simulink library "xbsIndex_r4"  (Simulink 7.1)
(part 8 of 9)

      |     e = regexprep(lasterr, '\n', '\nError: ');
      |     disp(['Error: While running MaskInit code on block ' tmp_gcb ': ' e]);
      |     error(e);
      |   end
      | end
      settings: AttributesFormatString=<< %<shared_memory_name> >>  CopyFcn=xlBlockMoveCallback(gcbh);  DeleteFcn=xlDestroyGui(gcbh);  ModelCloseFcn=xlDestroyGui(gcbh);  PreSaveFcn=xlBlockPreSaveCallback(gcbh);  PostSaveFcn=xlBlockPostSaveCallback(gcbh);  DestroyFcn=xlDestroyGui(gcbh);  OpenFcn=xlOpenGui(gcbh, 'tofifo_gui.xml', @tofifoenablement, @xlDatatypeAction)  CloseFcn=xlDestroyGui(gcbh);  MoveFcn=xlBlockMoveCallback(gcbh);
      mask Help: eval('');xlDoc('-book','sysgen','-topic','To_FIFO');
      mask StyleString: edit,edit,edit,popup(Locally owned|Owned elsewhere),edit,popup(Standard_FIFO|First_Word_Fall_Through),edit,popup(16|32|64|128|256|512|1K|2K|4K|8K|16K|32K|64K|128K|256K),edit,popup(1|2|3|4|5|6|7|8|9|10|11|12|13|14|15|16|17|18),edit,checkbox,edit,checkbox,edit,checkbox,popup(Fixed-point|Floating-point),edit,popup(Signed  (2's comp)|Unsigned|Floating-point),edit,edit,edit,popup(Single),edit,checkbox,edit,popup(Block RAM|Distributed RAM),edit,checkbox,edit,edit,edit,edit,edit,edit,edit,edit,edit
      mask Display:
      | fprintf('','COMMENT: begin icon graphics');
      | patch([0 80 80 0 0 ],[0 0 91 91 0 ],[0.77 0.82 0.91 ]);
      | plot([0 80 80 0 0 ],[0 0 91 91 0 ]);
      | patch([15.525 31.42 42.42 53.42 64.42 42.42 26.525 15.525 ],[57.21 57.21 68.21 57.21 68.21 68.21 68.21 57.21 ],[1 1 1 ]);
      | patch([26.525 42.42 31.42 15.525 26.525 ],[46.21 46.21 57.21 57.21 46.21 ],[0.931 0.946 0.973 ]);
      | patch([15.525 31.42 42.42 26.525 15.525 ],[35.21 35.21 46.21 46.21 35.21 ],[1 1 1 ]);
      | patch([26.525 64.42 53.42 42.42 31.42 15.525 26.525 ],[24.21 24.21 35.21 24.21 35.21 35.21 24.21 ],[0.931 0.946 0.973 ]);
      | fprintf('','COMMENT: end icon graphics');
      | fprintf('','COMMENT: begin icon text');
      | color('black');port_label('input',1,'data_in');
      | color('black');port_label('input',2,'we');
      | color('black');port_label('output',1,'%full');
      | color('black');port_label('output',2,'full');
      | fprintf('','COMMENT: end icon text');
  To Register : S-Function  LoadFcn=xlBlockLoadCallback(gcbh);  FunctionName=sysgen  Parameters=ptable_  EnableBusSupport=off  mask(Xilinx Shared Memory Based To Register Block){infoedit=Register block that writes data to a shared memory register.  Delay of one sample period., shared_memory_name='Bar', init=0, ownership_sgadvanced=, ownership=Locally owned and initialized, explicit_data_type_sgadvanced=, explicit_data_type=off, gui_display_data_type=Fixed-point, arith_type_sgadvanced=, arith_type=Signed  (2's comp), n_bits=16, bin_pt=14, preci_type_sgadvanced=, preci_type=Single, dbl_ovrd_sgadvanced=, dbl_ovrd=off, xl_use_area_sgadvanced=, xl_use_area=off, xl_area=[0,0,0,0,0,0,0], has_advanced_control=0, sggui_pos=-1,-1,-1,-1, block_type=toreg, block_version=, sg_icon_stat=60,56,2,1,white,blue,0,10ab453e,right,,[ ],[ ], sg_mask_display=|, sg_list_contents=, sg_blockgui_xml=}
      mask sg_mask_display=|
      | fprintf('','COMMENT: begin icon graphics');
      | patch([0 60 60 0 0 ],[0 0 56 56 0 ],[0.77 0.82 0.91 ]);
      | plot([0 60 60 0 0 ],[0 0 56 56 0 ]);
      | patch([12.2 23.76 31.76 39.76 47.76 31.76 20.2 12.2 ],[36.88 36.88 44.88 36.88 44.88 44.88 44.88 36.88 ],[1 1 1 ]);
      | patch([20.2 31.76 23.76 12.2 20.2 ],[28.88 28.88 36.88 36.88 28.88 ],[0.931 0.946 0.973 ]);
      | patch([12.2 23.76 31.76 20.2 12.2 ],[20.88 20.88 28.88 28.88 20.88 ],[1 1 1 ]);
      | patch([20.2 47.76 39.76 31.76 23.76 12.2 20.2 ],[12.88 12.88 20.88 12.88 20.88 20.88 12.88 ],[0.931 0.946 0.973 ]);
      | fprintf('','COMMENT: end icon graphics');
      | fprintf('','COMMENT: begin icon text');
      | color('black');port_label('input',1,'din');
      | color('black');port_label('input',2,'en');
      | color('black');port_label('output',1,'dout');
      | fprintf('','COMMENT: end icon text');
      mask prompts: infoedit ""; shared_memory_name "Shared memory name"; init "Initial value"; ownership_sgadvanced ""; ownership "Ownership and initialization"; explicit_data_type_sgadvanced ""; explicit_data_type "Specify explicit output type"; gui_display_data_type ""; arith_type_sgadvanced ""; arith_type "Arithmetic type"; n_bits "Number of bits"; bin_pt "Binary point"; preci_type_sgadvanced ""; preci_type ""; dbl_ovrd_sgadvanced ""; dbl_ovrd "Override with doubles"; xl_use_area_sgadvanced ""; xl_use_area "Define FPGA area for resource estimation"; xl_area "FPGA area [slices, FFs, BRAMs, LUTs, IOBs, emb. mults, TBUFs]"; has_advanced_control ""; sggui_pos ""; block_type ""; block_version ""; sg_icon_stat ""; sg_mask_display ""; sg_list_contents ""; sg_blockgui_xml ""
      mask help: Register block that writes data to a shared memory register. Delay of one sample period.
      mask init:
      | try
      |   tmp_gcb = gcb;
      |   tmp_gcbh = gcbh;
      |   if (strcmp('SysGenIndex',get_param(bdroot(tmp_gcbh),'tag')) && ~isempty(regexp(bdroot(tmp_gcb), '^xbs', 'once')))
      |     return;
      |   end;
      |   xlMungeMaskParams;
      |   block_config = 'sysgen_blockset:toreg_config';
      | 
      |   block_type='toreg';
      | 
      |   serialized_declarations = '{''arith_type''=>''Int'',''bin_pt''=>''Int'',''dbl_ovrd''=>''Int'',''explicit_data_type''=>''Int'',''gui_display_data_type''=>''Int'',''init''=>''Double'',''n_bits''=>''Int'',''ownership''=>''Int'',''preci_type''=>''Int'',''shared_memory_name''=>''String'',''block_type''=>''String''}';
      |   ptable_ = xlblockprep(get_param(tmp_gcb, 'MaskWSVariables'));
      |   try
      |     xlBlockMoveCallback(tmp_gcbh);
      |   catch 
      |      clear global xl_updateicon_recursion_guard;
      |   end;
      | catch
      |   global dbgsysgen;
      |   if(~isempty(dbgsysgen) && dbgsysgen)
      |     e = regexprep(lasterr, '\n', '\nError: ');
      |     disp(['Error: While running MaskInit code on block ' tmp_gcb ': ' e]);
      |     error(e);
      |   end
      | end
      settings: AttributesFormatString=<< %<shared_memory_name> >>  CopyFcn=xlBlockMoveCallback(gcbh);  DeleteFcn=xlDestroyGui(gcbh);  ModelCloseFcn=xlDestroyGui(gcbh);  PreSaveFcn=xlBlockPreSaveCallback(gcbh);  PostSaveFcn=xlBlockPostSaveCallback(gcbh);  DestroyFcn=xlDestroyGui(gcbh);  OpenFcn=xlOpenGui(gcbh, 'toreg_gui.xml', @toregenablement, @xlDatatypeAction)  CloseFcn=xlDestroyGui(gcbh);  MoveFcn=xlBlockMoveCallback(gcbh);
      mask Help: eval('');xlDoc('-book','sysgen','-topic','To_Register');
      mask StyleString: edit,edit,edit,edit,popup(Locally owned and initialized|Owned and initialized elsewhere),edit,checkbox,popup(Fixed-point|Floating-point),edit,popup(Signed  (2's comp)|Unsigned|Floating-point),edit,edit,edit,popup(Single),edit,checkbox,edit,checkbox,edit,edit,edit,edit,edit,edit,edit,edit,edit
      mask Display:
      | fprintf('','COMMENT: begin icon graphics');
      | patch([0 60 60 0 0 ],[0 0 56 56 0 ],[0.77 0.82 0.91 ]);
      | plot([0 60 60 0 0 ],[0 0 56 56 0 ]);
      | patch([12.2 23.76 31.76 39.76 47.76 31.76 20.2 12.2 ],[36.88 36.88 44.88 36.88 44.88 44.88 44.88 36.88 ],[1 1 1 ]);
      | patch([20.2 31.76 23.76 12.2 20.2 ],[28.88 28.88 36.88 36.88 28.88 ],[0.931 0.946 0.973 ]);
      | patch([12.2 23.76 31.76 20.2 12.2 ],[20.88 20.88 28.88 28.88 20.88 ],[1 1 1 ]);
      | patch([20.2 47.76 39.76 31.76 23.76 12.2 20.2 ],[12.88 12.88 20.88 12.88 20.88 20.88 12.88 ],[0.931 0.946 0.973 ]);
      | fprintf('','COMMENT: end icon graphics');
      | fprintf('','COMMENT: begin icon text');
      | color('black');port_label('input',1,'din');
      | color('black');port_label('input',2,'en');
      | color('black');port_label('output',1,'dout');
      | fprintf('','COMMENT: end icon text');
  Toolbar : S-Function  FunctionName=xlpermissive  Parameters=''  EnableBusSupport=off  mask(Xilinx Toolbar Block){infoedit=Toolbar, func=xltoolbar, ShowPortLabels=, has_advanced_control=0, sggui_pos=-1,-1,-1,-1, block_type=toolbar, block_version=, sg_icon_stat=50,54,-1,-1,blue,white,0,07734,right,,[ ],[ ], sg_mask_display=|, sg_list_contents=, sg_blockgui_xml=}
      mask sg_mask_display=|
      | fprintf('','COMMENT: begin icon graphics');
      | patch([0 50 50 0 0 ],[0 0 54 54 0 ],[1 1 1 ]);
      | plot([0 50 50 0 0 ],[0 0 54 54 0 ]);
      | patch([9.425 19.54 26.54 33.54 40.54 26.54 16.425 9.425 ],[34.77 34.77 41.77 34.77 41.77 41.77 41.77 34.77 ],[0.839 0.874 0.937 ]);
      | patch([16.425 26.54 19.54 9.425 16.425 ],[27.77 27.77 34.77 34.77 27.77 ],[0.77 0.82 0.91 ]);
      | patch([9.425 19.54 26.54 16.425 9.425 ],[20.77 20.77 27.77 27.77 20.77 ],[0.839 0.874 0.937 ]);
      | patch([16.425 40.54 33.54 26.54 19.54 9.425 16.425 ],[13.77 13.77 20.77 13.77 20.77 20.77 13.77 ],[0.77 0.82 0.91 ]);
      | fprintf('','COMMENT: end icon graphics');
      | fprintf('','COMMENT: begin icon text');
      | fprintf('','COMMENT: end icon text');
      mask prompts: infoedit ""; func "Launch function"; ShowPortLabels ""; has_advanced_control ""; sggui_pos ""; block_type ""; block_version ""; sg_icon_stat ""; sg_mask_display ""; sg_list_contents ""; sg_blockgui_xml ""
      mask help: Toolbar
      mask init:
      | try
      |   tmp_gcb = gcb;
      |   tmp_gcbh = gcbh;
      |   if (strcmp('SysGenIndex',get_param(bdroot(tmp_gcbh),'tag')) && ~isempty(regexp(bdroot(tmp_gcb), '^xbs', 'once')))
      |     return;
      |   end;
      |   xlMungeMaskParams;
      | 
      |   block_type='toolbar';
      | 
      |   serialized_declarations = '{''block_type''=>''String''}';
      |   ptable_ = xlblockprep(get_param(tmp_gcb, 'MaskWSVariables'));
      |   try
      |     xlBlockMoveCallback(tmp_gcbh);
      |   catch 
      |      clear global xl_updateicon_recursion_guard;
      |   end;
      | catch
      |   global dbgsysgen;
      |   if(~isempty(dbgsysgen) && dbgsysgen)
      |     e = regexprep(lasterr, '\n', '\nError: ');
      |     disp(['Error: While running MaskInit code on block ' tmp_gcb ': ' e]);
      |     error(e);
      |   end
      | end
      settings: CopyFcn=xlBlockMoveCallback(gcbh);  OpenFcn=xltoolbar;  MoveFcn=xlBlockMoveCallback(gcbh);
      mask Help: eval('');xlDoc('-book','sysgen','-topic','Toolbar');
      mask Display:
      | fprintf('','COMMENT: begin icon graphics');
      | patch([0 50 50 0 0 ],[0 0 54 54 0 ],[1 1 1 ]);
      | plot([0 50 50 0 0 ],[0 0 54 54 0 ]);
      | patch([9.425 19.54 26.54 33.54 40.54 26.54 16.425 9.425 ],[34.77 34.77 41.77 34.77 41.77 41.77 41.77 34.77 ],[0.839 0.874 0.937 ]);
      | patch([16.425 26.54 19.54 9.425 16.425 ],[27.77 27.77 34.77 34.77 27.77 ],[0.77 0.82 0.91 ]);
      | patch([9.425 19.54 26.54 16.425 9.425 ],[20.77 20.77 27.77 27.77 20.77 ],[0.839 0.874 0.937 ]);
      | patch([16.425 40.54 33.54 26.54 19.54 9.425 16.425 ],[13.77 13.77 20.77 13.77 20.77 20.77 13.77 ],[0.77 0.82 0.91 ]);
      | fprintf('','COMMENT: end icon graphics');
      | fprintf('','COMMENT: begin icon text');
      | fprintf('','COMMENT: end icon text');
  Up Sample : S-Function  LoadFcn=xlBlockLoadCallback(gcbh);  FunctionName=sysgen  Parameters=ptable_  EnableBusSupport=off  mask(Xilinx Up Sampler Block){infoedit=Up samples input data.  Inserted values  can be zeros or copies of the most recent input sample.<br><br>Hardware notes: No hardware is needed if inserted values are copies of the input sample; otherwise, a mux and single bit flip-flop are used., sample_ratio=2, copy_samples_sgadvanced=, copy_samples=off, en_sgadvanced=, en=off, latency=0, dbl_ovrd_sgadvanced=, dbl_ovrd=off, xl_use_area_sgadvanced=, xl_use_area=off, xl_area=[0,0,0,0,0,0,0], has_advanced_control=0, sggui_pos=-1,-1,-1,-1, block_type=usamp, block_version=, sg_icon_stat=60,54,1,1,white,blue,0,cf641474,right,,[ ],[ ], sg_mask_display=|, sg_list_contents=, sg_blockgui_xml=}
      mask sg_mask_display=|
      | fprintf('','COMMENT: begin icon graphics');
      | patch([0 60 60 0 0 ],[0 0 54 54 0 ],[0.77 0.82 0.91 ]);
      | plot([0 60 60 0 0 ],[0 0 54 54 0 ]);
      | patch([14.425 24.54 31.54 38.54 45.54 31.54 21.425 14.425 ],[34.77 34.77 41.77 34.77 41.77 41.77 41.77 34.77 ],[1 1 1 ]);
      | patch([21.425 31.54 24.54 14.425 21.425 ],[27.77 27.77 34.77 34.77 27.77 ],[0.931 0.946 0.973 ]);
      | patch([14.425 24.54 31.54 21.425 14.425 ],[20.77 20.77 27.77 27.77 20.77 ],[1 1 1 ]);
      | patch([21.425 45.54 38.54 31.54 24.54 14.425 21.425 ],[13.77 13.77 20.77 13.77 20.77 20.77 13.77 ],[0.931 0.946 0.973 ]);
      | fprintf('','COMMENT: end icon graphics');
      | fprintf('','COMMENT: begin icon text');
      |
      |
      | color('black');disp('{\fontsize{14pt}\bf\uparrow}2','texmode','on');
      | fprintf('','COMMENT: end icon text');
      mask prompts: infoedit ""; sample_ratio "Sampling rate (number of output samples per input sample)"; copy_samples_sgadvanced ""; copy_samples "Copy samples (otherwise zeros are inserted)"; en_sgadvanced ""; en "Provide enable port"; dbl_ovrd_sgadvanced ""; dbl_ovrd "Override with doubles"; xl_use_area_sgadvanced ""; xl_use_area "Define FPGA area for resource estimation"; xl_area "FPGA area [slices, FFs, BRAMs, LUTs, IOBs, emb. mults, TBUFs]"; has_advanced_control ""; sggui_pos ""; block_type ""; block_version ""; sg_icon_stat ""; sg_mask_display ""; sg_list_contents ""; sg_blockgui_xml ""
      mask help:
      | Up samples input data.  Inserted values  can be zeros or copies of the most recent input sample.
      |
      | Hardware notes: No hardware is needed if inserted values are copies of the input sample; otherwise, a mux and single bit flip-flop are used.
      mask init:
      | try
      |   tmp_gcb = gcb;
      |   tmp_gcbh = gcbh;
      |   if (strcmp('SysGenIndex',get_param(bdroot(tmp_gcbh),'tag')) && ~isempty(regexp(bdroot(tmp_gcb), '^xbs', 'once')))
      |     return;
      |   end;
      |   xlMungeMaskParams;
      |   block_config = 'sysgen_blockset:Upsample_config';
      | 
      |   block_type='usamp';
      | 
      |   serialized_declarations = '{''copy_samples''=>''Int'',''en''=>''Int'',''latency''=>''Int'',''sample_ratio''=>''Int'',''sim_engine''=>''Int'',''sysgen_root''=>''String'',''block_type''=>''String''}';
      |   xlusamp_init();
      |   ptable_ = xlblockprep(get_param(tmp_gcb, 'MaskWSVariables'));
      |   try
      |     xlBlockMoveCallback(tmp_gcbh);
      |   catch 
      |      clear global xl_updateicon_recursion_guard;
      |   end;
      | catch
      |   global dbgsysgen;
      |   if(~isempty(dbgsysgen) && dbgsysgen)
      |     e = regexprep(lasterr, '\n', '\nError: ');
      |     disp(['Error: While running MaskInit code on block ' tmp_gcb ': ' e]);
      |     error(e);
      |   end
      | end
      settings: CopyFcn=xlBlockMoveCallback(gcbh);  DeleteFcn=xlDestroyGui(gcbh);  ModelCloseFcn=xlDestroyGui(gcbh);  PreSaveFcn=xlBlockPreSaveCallback(gcbh);  PostSaveFcn=xlBlockPostSaveCallback(gcbh);  DestroyFcn=xlDestroyGui(gcbh);  OpenFcn=xlOpenGui(gcbh, 'usamp_gui.xml', @xlmagicenablement, -1)  CloseFcn=xlDestroyGui(gcbh);  MoveFcn=xlBlockMoveCallback(gcbh);
      mask Help: eval('');xlDoc('-book','sysgen','-topic','Up_Sample');
      mask Display:
      | fprintf('','COMMENT: begin icon graphics');
      | patch([0 60 60 0 0 ],[0 0 54 54 0 ],[0.77 0.82 0.91 ]);
      | plot([0 60 60 0 0 ],[0 0 54 54 0 ]);
      | patch([14.425 24.54 31.54 38.54 45.54 31.54 21.425 14.425 ],[34.77 34.77 41.77 34.77 41.77 41.77 41.77 34.77 ],[1 1 1 ]);
      | patch([21.425 31.54 24.54 14.425 21.425 ],[27.77 27.77 34.77 34.77 27.77 ],[0.931 0.946 0.973 ]);
      | patch([14.425 24.54 31.54 21.425 14.425 ],[20.77 20.77 27.77 27.77 20.77 ],[1 1 1 ]);
      | patch([21.425 45.54 38.54 31.54 24.54 14.425 21.425 ],[13.77 13.77 20.77 13.77 20.77 20.77 13.77 ],[0.931 0.946 0.973 ]);
      | fprintf('','COMMENT: end icon graphics');
      | fprintf('','COMMENT: begin icon text');
      | 
      | 
      | color('black');disp('{\fontsize{14pt}\bf\uparrow}2','texmode','on');
      | fprintf('','COMMENT: end icon text');
  "VDMA Interface 4.0 " : S-Function  LoadFcn=xlBlockLoadCallback(gcbh);  FunctionName=sysgen  Parameters=ptable_  EnableBusSupport=off  mask(Xilinx VDMA Interface Block){infoedit=This is a bit-accurate simulation model for multiple AXI VDMA external memory interfaces.  Netlisting will generate the port interface that can be attached to the VDMA IP.  This block is currently in beta., c_mem_size_sgadvanced=, c_mem_size=64MB, c_number_of_vdma_if_sgadvanced=, c_number_of_vdma_if=1, c_stream_if_configuration_1_sgadvanced=, c_stream_if_configuration_1=Master/Slave, c_no_of_frames_1=3, c_use_fsync_1_sgadvanced=, c_use_fsync_1=off, c_flush_on_fsync_1_sgadvanced=, c_flush_on_fsync_1=off, c_use_sg_engine_1_sgadvanced=, c_use_sg_engine_1=off, c_video_prm_read_1_sgadvanced=, c_video_prm_read_1=on, c_m_axis_mm2s_data_width_1_sgadvanced=, c_m_axis_mm2s_data_width_1=32, c_mm2s_linebuffer_depth_1_sgadvanced=, c_mm2s_linebuffer_depth_1=0, c_mm2s_linebuffer_threshold_1=1, c_s_axis_s2mm_data_width_1_sgadvanced=, c_s_axis_s2mm_data_width_1=32, c_s2mm_linebuffer_depth_1_sgadvanced=, c_s2mm_linebuffer_depth_1=0, c_s2mm_linebuffer_threshold_1=1, c_stream_if_configuration_2_sgadvanced=, c_stream_if_configuration_2=Master/Slave, c_no_of_frames_2=3, c_use_fsync_2_sgadvanced=, c_use_fsync_2=off, c_flush_on_fsync_2_sgadvanced=, c_flush_on_fsync_2=off, c_use_sg_engine_2_sgadvanced=, c_use_sg_engine_2=off, c_video_prm_read_2_sgadvanced=, c_video_prm_read_2=on, c_m_axis_mm2s_data_width_2_sgadvanced=, c_m_axis_mm2s_data_width_2=32, c_mm2s_linebuffer_depth_2_sgadvanced=, c_mm2s_linebuffer_depth_2=0, c_mm2s_linebuffer_threshold_2=1, c_s_axis_s2mm_data_width_2_sgadvanced=, c_s_axis_s2mm_data_width_2=32, c_s2mm_linebuffer_depth_2_sgadvanced=, c_s2mm_linebuffer_depth_2=0, c_s2mm_linebuffer_threshold_2=1, c_stream_if_configuration_3_sgadvanced=, c_stream_if_configuration_3=Master/Slave, c_no_of_frames_3=3, c_use_fsync_3_sgadvanced=, c_use_fsync_3=off, c_flush_on_fsync_3_sgadvanced=, c_flush_on_fsync_3=off, c_use_sg_engine_3_sgadvanced=, c_use_sg_engine_3=off, c_video_prm_read_3_sgadvanced=, c_video_prm_read_3=on, c_m_axis_mm2s_data_width_3_sgadvanced=, c_m_axis_mm2s_data_width_3=32, c_mm2s_linebuffer_depth_3_sgadvanced=, c_mm2s_linebuffer_depth_3=0, c_mm2s_linebuffer_threshold_3=1, c_s_axis_s2mm_data_width_3_sgadvanced=, c_s_axis_s2mm_data_width_3=32, c_s2mm_linebuffer_depth_3_sgadvanced=, c_s2mm_linebuffer_depth_3=0, c_s2mm_linebuffer_threshold_3=1, c_stream_if_configuration_4_sgadvanced=, c_stream_if_configuration_4=Master/Slave, c_no_of_frames_4=3, c_use_fsync_4_sgadvanced=, c_use_fsync_4=off, c_flush_on_fsync_4_sgadvanced=, c_flush_on_fsync_4=off, c_use_sg_engine_4_sgadvanced=, c_use_sg_engine_4=off, c_video_prm_read_4_sgadvanced=, c_video_prm_read_4=on, c_m_axis_mm2s_data_width_4_sgadvanced=, c_m_axis_mm2s_data_width_4=32, c_mm2s_linebuffer_depth_4_sgadvanced=, c_mm2s_linebuffer_depth_4=0, c_mm2s_linebuffer_threshold_4=1, c_s_axis_s2mm_data_width_4_sgadvanced=, c_s_axis_s2mm_data_width_4=32, c_s2mm_linebuffer_depth_4_sgadvanced=, c_s2mm_linebuffer_depth_4=0, c_s2mm_linebuffer_threshold_4=1, simulation_model='emi:EMIModel', has_advanced_control=0, sggui_pos=-1,-1,-1,-1, block_type=vdma, block_version=, sg_icon_stat=335,744,14,19,white,yellow,0,358287e6,right,,[2 2 2 2 2 2 2 2 3 3 3 3 4 1 ],[2 2 2 2 2 2 2 2 3 4 4 4 4 1 1 1 1 1 1 ], sg_mask_display=|, sg_list_contents=, sg_blockgui_xml=}
      mask sg_mask_display=|
      | fprintf('','COMMENT: begin icon graphics');
      | patch([0 0 5 5 ],[744 323 323 744 ],[7.375000e-001 7.225000e-001 5.125000e-001 ]);
      | patch([0 0 5 5 ],[306 103 103 306 ],[5.250000e-001 5.150000e-001 3.750000e-001 ]);
      | patch([0 0 5 5 ],[86 48 48 86 ],[3.125000e-001 3.075000e-001 2.375000e-001 ]);
      | patch([0 0 5 5 ],[31 -7 -7 31 ],[9.500000e-001 9.300000e-001 6.500000e-001 ]);
      | patch([330 330 335 335 ],[744 438 438 744 ],[7.375000e-001 7.225000e-001 5.125000e-001 ]);
      | patch([330 330 335 335 ],[426 398 398 426 ],[5.250000e-001 5.150000e-001 3.750000e-001 ]);
      | patch([330 330 335 335 ],[386 238 238 386 ],[3.125000e-001 3.075000e-001 2.375000e-001 ]);
      | patch([330 330 335 335 ],[226 -2 -2 226 ],[9.500000e-001 9.300000e-001 6.500000e-001 ]);
      | patch([5 329 329 5 5 ],[0 0 744 744 0 ],[9.500000e-001 9.300000e-001 6.500000e-001 ]);
      | plot([5 329 329 5 5 ],[0 0 744 744 0 ]);
      |
      |
      | patch([62.425 130.34 177.34 224.34 271.34 177.34 109.425 62.425 ],[424.17 424.17 471.17 424.17 471.17 471.17 471.17 424.17 ],[1 1 1 ]);
      | patch([109.425 177.34 130.34 62.425 109.425 ],[377.17 377.17 424.17 424.17 377.17 ],[0.985 0.979 0.895 ]);
      | patch([62.425 130.34 177.34 109.425 62.425 ],[330.17 330.17 377.17 377.17 330.17 ],[1 1 1 ]);
      | patch([109.425 271.34 224.34 177.34 130.34 62.425 109.425 ],[283.17 283.17 330.17 283.17 330.17 330.17 283.17 ],[0.985 0.979 0.895 ]);
      | fprintf('','COMMENT: end icon graphics');
      | fprintf('','COMMENT: begin icon text');
      | color('black');port_label('input',1,'  vdma_1_s_axi_lite_awvalid  ');
      | color('black');port_label('input',2,'  vdma_1_s_axi_lite_awaddr  ');
      | color('black');port_label('input',3,'  vdma_1_s_axi_lite_wvalid  ');
      | color('black');port_label('input',4,'  vdma_1_s_axi_lite_wdata  ');
      | color('black');port_label('input',5,'  vdma_1_s_axi_lite_bready  ');
      | color('black');port_label('input',6,'  vdma_1_s_axi_lite_arvalid  ');
      | color('black');port_label('input',7,'  vdma_1_s_axi_lite_araddr  ');
      | color('black');port_label('input',8,'  vdma_1_s_axi_lite_rready  ');
      | color('black');port_label('input',9,'  vdma_1_s_axis_s2mm_tdata  ');
      | color('black');port_label('input',10,'  vdma_1_s_axis_s2mm_tkeep  ');
      | color('black');port_label('input',11,'  vdma_1_s_axis_s2mm_tvalid  ');
      | color('black');port_label('input',12,'  vdma_1_s_axis_s2mm_tlast  ');
      | color('black');port_label('input',13,'  vdma_1_m_axis_mm2s_tready  ');
      | color('black');port_label('input',14,'  vdma_1_axi_resetn  ');
      | color('black');port_label('output',1,'  vdma_1_s_axi_lite_awready  ');
      | color('black');port_label('output',2,'  vdma_1_s_axi_lite_wready  ');
      | color('black');port_label('output',3,'  vdma_1_s_axi_lite_bresp  ');
      | color('black');port_label('output',4,'  vdma_1_s_axi_lite_bvalid  ');
      | color('black');port_label('output',5,'  vdma_1_s_axi_lite_arready  ');
      | color('black');port_label('output',6,'  vdma_1_s_axi_lite_rvalid  ');
      | color('black');port_label('output',7,'  vdma_1_s_axi_lite_rdata  ');
      | color('black');port_label('output',8,'  vdma_1_s_axi_lite_rresp  ');
      | color('black');port_label('output',9,'  vdma_1_s_axis_s2mm_tready  ');
      | color('black');port_label('output',10,'  vdma_1_m_axis_mm2s_tdata  ');
      | color('black');port_label('output',11,'  vdma_1_m_axis_mm2s_tkeep  ');
      | color('black');port_label('output',12,'  vdma_1_m_axis_mm2s_tvalid  ');
      | color('black');port_label('output',13,'  vdma_1_m_axis_mm2s_tlast  ');
      | color('black');port_label('output',14,'  vdma_1_mm2s_introut  ');
      | color('black');port_label('output',15,'  vdma_1_mm2s_fsync_out  ');
      | color('black');port_label('output',16,'  vdma_1_mm2s_prmtr_update  ');
      | color('black');port_label('output',17,'  vdma_1_s2mm_introut  ');
      | color('black');port_label('output',18,'  vdma_1_s2mm_fsync_out  ');
      | color('black');port_label('output',19,'  vdma_1_s2mm_prmtr_update  ');
      | fprintf('','COMMENT: end icon text');
      mask prompts: infoedit ""; c_mem_size_sgadvanced ""; c_mem_size "Memory size"; c_number_of_vdma_if_sgadvanced ""; c_number_of_vdma_if "Number of VDMA interfaces"; c_stream_if_configuration_1_sgadvanced ""; c_stream_if_configuration_1 "Stream interface"; c_no_of_frames_1 "Number of frame stores [1..16]"; c_use_fsync_1_sgadvanced ""; c_use_fsync_1 "Use external frame sync"; c_flush_on_fsync_1_sgadvanced ""; c_flush_on_fsync_1 "Flush on frame sync"; c_use_sg_engine_1_sgadvanced ""; c_use_sg_engine_1 "Use Scatter Gather Engine"; c_video_prm_read_1_sgadvanced ""; c_video_prm_read_1 "Use Video Parameter Read for Direct Mode"; c_m_axis_mm2s_data_width_1_sgadvanced ""; c_m_axis_mm2s_data_width_1 "Data width"; c_mm2s_linebuffer_depth_1_sgadvanced ""; c_mm2s_linebuffer_depth_1 "Depth"; c_mm2s_linebuffer_threshold_1 "Almost empty threshold [1..65536]"; c_s_axis_s2mm_data_width_1_sgadvanced ""; c_s_axis_s2mm_data_width_1 "Data width"; c_s2mm_linebuffer_depth_1_sgadvanced ""; c_s2mm_linebuffer_depth_1 "Depth"; c_s2mm_linebuffer_threshold_1 "Almost full threshold [1..65536]"; c_stream_if_configuration_2_sgadvanced ""; c_stream_if_configuration_2 "Stream interface"; c_no_of_frames_2 "Number of frame stores [1..16]"; c_use_fsync_2_sgadvanced ""; c_use_fsync_2 "Use external frame sync"; c_flush_on_fsync_2_sgadvanced ""; c_flush_on_fsync_2 "Flush on frame sync"; c_use_sg_engine_2_sgadvanced ""; c_use_sg_engine_2 "Use Scatter Gather Engine"; c_video_prm_read_2_sgadvanced ""; c_video_prm_read_2 "Use Video Parameter Read for Direct Mode"; c_m_axis_mm2s_data_width_2_sgadvanced ""; c_m_axis_mm2s_data_width_2 "Data width"; c_mm2s_linebuffer_depth_2_sgadvanced ""; c_mm2s_linebuffer_depth_2 "Depth"; c_mm2s_linebuffer_threshold_2 "Almost empty threshold [1..65536]"; c_s_axis_s2mm_data_width_2_sgadvanced ""; c_s_axis_s2mm_data_width_2 "Data width"; c_s2mm_linebuffer_depth_2_sgadvanced ""; c_s2mm_linebuffer_depth_2 "Depth"; c_s2mm_linebuffer_threshold_2 "Almost full threshold [1..65536]"; c_stream_if_configuration_3_sgadvanced ""; c_stream_if_configuration_3 "Stream interface"; c_no_of_frames_3 "Number of frame stores [1..16]"; c_use_fsync_3_sgadvanced ""; c_use_fsync_3 "Use external frame sync"; c_flush_on_fsync_3_sgadvanced ""; c_flush_on_fsync_3 "Flush on frame sync"; c_use_sg_engine_3_sgadvanced ""; c_use_sg_engine_3 "Use Scatter Gather Engine"; c_video_prm_read_3_sgadvanced ""; c_video_prm_read_3 "Use Video Parameter Read for Direct Mode"; c_m_axis_mm2s_data_width_3_sgadvanced ""; c_m_axis_mm2s_data_width_3 "Data width"; c_mm2s_linebuffer_depth_3_sgadvanced ""; c_mm2s_linebuffer_depth_3 "Depth"; c_mm2s_linebuffer_threshold_3 "Almost empty threshold [1..65536]"; c_s_axis_s2mm_data_width_3_sgadvanced ""; c_s_axis_s2mm_data_width_3 "Data width"; c_s2mm_linebuffer_depth_3_sgadvanced ""; c_s2mm_linebuffer_depth_3 "Depth"; c_s2mm_linebuffer_threshold_3 "Almost full threshold [1..65536]"; c_stream_if_configuration_4_sgadvanced ""; c_stream_if_configuration_4 "Stream interface"; c_no_of_frames_4 "Number of frame stores [1..16]"; c_use_fsync_4_sgadvanced ""; c_use_fsync_4 "Use external frame sync"; c_flush_on_fsync_4_sgadvanced ""; c_flush_on_fsync_4 "Flush on frame sync"; c_use_sg_engine_4_sgadvanced ""; c_use_sg_engine_4 "Use Scatter Gather Engine"; c_video_prm_read_4_sgadvanced ""; c_video_prm_read_4 "Use Video Parameter Read for Direct Mode"; c_m_axis_mm2s_data_width_4_sgadvanced ""; c_m_axis_mm2s_data_width_4 "Data width"; c_mm2s_linebuffer_depth_4_sgadvanced ""; c_mm2s_linebuffer_depth_4 "Depth"; c_mm2s_linebuffer_threshold_4 "Almost empty threshold [1..65536]"; c_s_axis_s2mm_data_width_4_sgadvanced ""; c_s_axis_s2mm_data_width_4 "Data width"; c_s2mm_linebuffer_depth_4_sgadvanced ""; c_s2mm_linebuffer_depth_4 "Depth"; c_s2mm_linebuffer_threshold_4 "Almost full threshold [1..65536]"; simulation_model ""; has_advanced_control ""; sggui_pos ""; block_type ""; block_version ""; sg_icon_stat ""; sg_mask_display ""; sg_list_contents ""; sg_blockgui_xml ""
      mask help: This is a bit-accurate simulation model for multiple AXI VDMA external memory interfaces. Netlisting will generate the port interface that can be attached to the VDMA IP. This block is currently in beta.
      mask init:
      | try
      |   tmp_gcb = gcb;
      |   tmp_gcbh = gcbh;
      |   if (strcmp('SysGenIndex',get_param(bdroot(tmp_gcbh),'tag')) && ~isempty(regexp(bdroot(tmp_gcb), '^xbs', 'once')))
      |     return;
      |   end;
      |   xlMungeMaskParams;
      |   block_config = 'emi:emi_all_interfaces_config';
      | 
      |   block_type='vdma';
      | 
      |   serialized_declarations = '{''c_flush_on_fsync_1''=>''Int'',''c_flush_on_fsync_2''=>''Int'',''c_flush_on_fsync_3''=>''Int'',''c_flush_on_fsync_4''=>''Int'',''c_m_axis_mm2s_data_width_1''=>''Int'',''c_m_axis_mm2s_data_width_2''=>''Int'',''c_m_axis_mm2s_data_width_3''=>''Int'',''c_m_axis_mm2s_data_width_4''=>''Int'',''c_mem_size''=>''Int'',''c_mm2s_linebuffer_depth_1''=>''Int'',''c_mm2s_linebuffer_depth_2''=>''Int'',''c_mm2s_linebuffer_depth_3''=>''Int'',''c_mm2s_linebuffer_depth_4''=>''Int'',''c_mm2s_linebuffer_threshold_1''=>''Int'',''c_mm2s_linebuffer_threshold_2''=>''Int'',''c_mm2s_linebuffer_threshold_3''=>''Int'',''c_mm2s_linebuffer_threshold_4''=>''Int'',''c_no_of_frames_1''=>''Int'',''c_no_of_frames_2''=>''Int'',''c_no_of_frames_3''=>''Int'',''c_no_of_frames_4''=>''Int'',''c_number_of_vdma_if''=>''Int'',''c_s2mm_linebuffer_depth_1''=>''Int'',''c_s2mm_linebuffer_depth_2''=>''Int'',''c_s2mm_linebuffer_depth_3''=>''Int'',''c_s2mm_linebuffer_depth_4''=>''Int'',''c_s2mm_linebuffer_threshold_1''=>''Int'',''c_s2mm_linebuffer_threshold_2''=>''Int'',''c_s2mm_linebuffer_threshold_3''=>''Int'',''c_s2mm_linebuffer_threshold_4''=>''Int'',''c_s_axis_s2mm_data_width_1''=>''Int'',''c_s_axis_s2mm_data_width_2''=>''Int'',''c_s_axis_s2mm_data_width_3''=>''Int'',''c_s_axis_s2mm_data_width_4''=>''Int'',''c_stream_if_configuration_1''=>''Int'',''c_stream_if_configuration_2''=>''Int'',''c_stream_if_configuration_3''=>''Int'',''c_stream_if_configuration_4''=>''Int'',''c_use_fsync_1''=>''Int'',''c_use_fsync_2''=>''Int'',''c_use_fsync_3''=>''Int'',''c_use_fsync_4''=>''Int'',''c_use_sg_engine_1''=>''Int'',''c_use_sg_engine_2''=>''Int'',''c_use_sg_engine_3''=>''Int'',''c_use_sg_engine_4''=>''Int'',''c_video_prm_read_1''=>''Int'',''c_video_prm_read_2''=>''Int'',''c_video_prm_read_3''=>''Int'',''c_video_prm_read_4''=>''Int'',''simulation_model''=>''String'',''block_type''=>''String''}';
      |   ptable_ = xlblockprep(get_param(tmp_gcb, 'MaskWSVariables'));
      |   try
      |     xlBlockMoveCallback(tmp_gcbh);
      |   catch 
      |      clear global xl_updateicon_recursion_guard;
      |   end;
      | catch
      |   global dbgsysgen;
      |   if(~isempty(dbgsysgen) && dbgsysgen)
      |     e = regexprep(lasterr, '\n', '\nError: ');
      |     disp(['Error: While running MaskInit code on block ' tmp_gcb ': ' e]);
      |     error(e);
      |   end
      | end
      settings: CopyFcn=xlBlockMoveCallback(gcbh);  DeleteFcn=xlDestroyGui(gcbh);  ModelCloseFcn=xlDestroyGui(gcbh);  PreSaveFcn=xlBlockPreSaveCallback(gcbh);  PostSaveFcn=xlBlockPostSaveCallback(gcbh);  DestroyFcn=xlDestroyGui(gcbh);  OpenFcn=xlOpenGui(gcbh, 'vdma_gui.xml', @xlEMIEnablement, @xlEMIaction)  CloseFcn=xlDestroyGui(gcbh);  MoveFcn=xlBlockMoveCallback(gcbh);
      mask Help: eval('');xlDoc('-book','sysgen','-topic','VDMA_Interface_4_0');
      mask StyleString: edit,edit,popup(16MB|32MB|64MB|128MB|256MB|512MB|1GB|2GB),edit,popup(1|2|3|4),edit,popup(Master/Slave|Master|Slave),edit,edit,checkbox,edit,checkbox,edit,checkbox,edit,checkbox,edit,popup(8|16|32|64|128|256|512|1024),edit,popup(0|1|2|4|8|16|32|64|128|256|512|1024|2048|4096|8192|16384|32768|65536),edit,edit,popup(8|16|32|64|128|256|512|1024),edit,popup(0|1|2|4|8|16|32|64|128|256|512|1024|2048|4096|8192|16384|32768|65536),edit,edit,popup(Master/Slave|Master|Slave),edit,edit,checkbox,edit,checkbox,edit,checkbox,edit,checkbox,edit,popup(8|16|32|64|128|256|512|1024),edit,popup(0|1|2|4|8|16|32|64|128|256|512|1024|2048|4096|8192|16384|32768|65536),edit,edit,popup(8|16|32|64|128|256|512|1024),edit,popup(0|1|2|4|8|16|32|64|128|256|512|1024|2048|4096|8192|16384|32768|65536),edit,edit,popup(Master/Slave|Master|Slave),edit,edit,checkbox,edit,checkbox,edit,checkbox,edit,checkbox,edit,popup(8|16|32|64|128|256|512|1024),edit,popup(0|1|2|4|8|16|32|64|128|256|512|1024|2048|4096|8192|16384|32768|65536),edit,edit,popup(8|16|32|64|128|256|512|1024),edit,popup(0|1|2|4|8|16|32|64|128|256|512|1024|2048|4096|8192|16384|32768|65536),edit,edit,popup(Master/Slave|Master|Slave),edit,edit,checkbox,edit,checkbox,edit,checkbox,edit,checkbox,edit,popup(8|16|32|64|128|256|512|1024),edit,popup(0|1|2|4|8|16|32|64|128|256|512|1024|2048|4096|8192|16384|32768|65536),edit,edit,popup(8|16|32|64|128|256|512|1024),edit,popup(0|1|2|4|8|16|32|64|128|256|512|1024|2048|4096|8192|16384|32768|65536),edit,edit,edit,edit,edit,edit,edit,edit,edit,edit
      mask Display:
      | fprintf('','COMMENT: begin icon graphics');
      | patch([0 0 5 5 ],[744 323 323 744 ],[7.375000e-001 7.225000e-001 5.125000e-001 ]);
      | patch([0 0 5 5 ],[306 103 103 306 ],[5.250000e-001 5.150000e-001 3.750000e-001 ]);
      | patch([0 0 5 5 ],[86 48 48 86 ],[3.125000e-001 3.075000e-001 2.375000e-001 ]);
      | patch([0 0 5 5 ],[31 -7 -7 31 ],[9.500000e-001 9.300000e-001 6.500000e-001 ]);
      | patch([330 330 335 335 ],[744 438 438 744 ],[7.375000e-001 7.225000e-001 5.125000e-001 ]);
      | patch([330 330 335 335 ],[426 398 398 426 ],[5.250000e-001 5.150000e-001 3.750000e-001 ]);
      | patch([330 330 335 335 ],[386 238 238 386 ],[3.125000e-001 3.075000e-001 2.375000e-001 ]);
      | patch([330 330 335 335 ],[226 -2 -2 226 ],[9.500000e-001 9.300000e-001 6.500000e-001 ]);
      | patch([5 329 329 5 5 ],[0 0 744 744 0 ],[9.500000e-001 9.300000e-001 6.500000e-001 ]);
      | plot([5 329 329 5 5 ],[0 0 744 744 0 ]);
      | 
      | 
      | patch([62.425 130.34 177.34 224.34 271.34 177.34 109.425 62.425 ],[424.17 424.17 471.17 424.17 471.17 471.17 471.17 424.17 ],[1 1 1 ]);
      | patch([109.425 177.34 130.34 62.425 109.425 ],[377.17 377.17 424.17 424.17 377.17 ],[0.985 0.979 0.895 ]);
      | patch([62.425 130.34 177.34 109.425 62.425 ],[330.17 330.17 377.17 377.17 330.17 ],[1 1 1 ]);
      | patch([109.425 271.34 224.34 177.34 130.34 62.425 109.425 ],[283.17 283.17 330.17 283.17 330.17 330.17 283.17 ],[0.985 0.979 0.895 ]);
      | fprintf('','COMMENT: end icon graphics');
      | fprintf('','COMMENT: begin icon text');
      | color('black');port_label('input',1,'  vdma_1_s_axi_lite_awvalid  ');
      | color('black');port_label('input',2,'  vdma_1_s_axi_lite_awaddr  ');
      | color('black');port_label('input',3,'  vdma_1_s_axi_lite_wvalid  ');
      | color('black');port_label('input',4,'  vdma_1_s_axi_lite_wdata  ');
      | color('black');port_label('input',5,'  vdma_1_s_axi_lite_bready  ');
      | color('black');port_label('input',6,'  vdma_1_s_axi_lite_arvalid  ');
      | color('black');port_label('input',7,'  vdma_1_s_axi_lite_araddr  ');
      | color('black');port_label('input',8,'  vdma_1_s_axi_lite_rready  ');
      | color('black');port_label('input',9,'  vdma_1_s_axis_s2mm_tdata  ');
      | color('black');port_label('input',10,'  vdma_1_s_axis_s2mm_tkeep  ');
      | color('black');port_label('input',11,'  vdma_1_s_axis_s2mm_tvalid  ');
      | color('black');port_label('input',12,'  vdma_1_s_axis_s2mm_tlast  ');
      | color('black');port_label('input',13,'  vdma_1_m_axis_mm2s_tready  ');
      | color('black');port_label('input',14,'  vdma_1_axi_resetn  ');
      | color('black');port_label('output',1,'  vdma_1_s_axi_lite_awready  ');
      | color('black');port_label('output',2,'  vdma_1_s_axi_lite_wready  ');
      | color('black');port_label('output',3,'  vdma_1_s_axi_lite_bresp  ');
      | color('black');port_label('output',4,'  vdma_1_s_axi_lite_bvalid  ');
      | color('black');port_label('output',5,'  vdma_1_s_axi_lite_arready  ');
      | color('black');port_label('output',6,'  vdma_1_s_axi_lite_rvalid  ');
      | color('black');port_label('output',7,'  vdma_1_s_axi_lite_rdata  ');
      | color('black');port_label('output',8,'  vdma_1_s_axi_lite_rresp  ');
      | color('black');port_label('output',9,'  vdma_1_s_axis_s2mm_tready  ');
      | color('black');port_label('output',10,'  vdma_1_m_axis_mm2s_tdata  ');
      | color('black');port_label('output',11,'  vdma_1_m_axis_mm2s_tkeep  ');
      | color('black');port_label('output',12,'  vdma_1_m_axis_mm2s_tvalid  ');
      | color('black');port_label('output',13,'  vdma_1_m_axis_mm2s_tlast  ');
      | color('black');port_label('output',14,'  vdma_1_mm2s_introut  ');
      | color('black');port_label('output',15,'  vdma_1_mm2s_fsync_out  ');
      | color('black');port_label('output',16,'  vdma_1_mm2s_prmtr_update  ');
      | color('black');port_label('output',17,'  vdma_1_s2mm_introut  ');
      | color('black');port_label('output',18,'  vdma_1_s2mm_fsync_out  ');
      | color('black');port_label('output',19,'  vdma_1_s2mm_prmtr_update  ');
      | fprintf('','COMMENT: end icon text');
  "VDMA Interface 5.0 " : S-Function  LoadFcn=xlBlockLoadCallback(gcbh);  FunctionName=sysgen  Parameters=ptable_  EnableBusSupport=off  mask(Xilinx VDMA Interface 5.0 Block){infoedit=This is a bit-accurate simulation model for multiple AXI VDMA external memory interfaces.  Netlisting will generate the port interface that can be attached to the VDMA IP.  This block is currently in beta., c_mem_size_sgadvanced=, c_mem_size=64MB, c_number_of_vdma_if_sgadvanced=, c_number_of_vdma_if=1, c_stream_if_configuration_1_sgadvanced=, c_stream_if_configuration_1=Master/Slave, c_no_of_frames_1=3, c_use_fsync_1_sgadvanced=, c_use_fsync_1=off, c_flush_on_fsync_1_sgadvanced=, c_flush_on_fsync_1=off, c_use_sg_engine_1_sgadvanced=, c_use_sg_engine_1=off, c_video_prm_read_1_sgadvanced=, c_video_prm_read_1=on, c_m_axis_mm2s_data_width_1_sgadvanced=, c_m_axis_mm2s_data_width_1=32, c_m_axis_mm2s_frame_sync_tuser_1_sgadvanced=, c_m_axis_mm2s_frame_sync_tuser_1=off, c_mm2s_linebuffer_depth_1_sgadvanced=, c_mm2s_linebuffer_depth_1=0, c_mm2s_linebuffer_threshold_1=1, c_s_axis_s2mm_data_width_1_sgadvanced=, c_s_axis_s2mm_data_width_1=32, c_s_axis_s2mm_frame_sync_tuser_1_sgadvanced=, c_s_axis_s2mm_frame_sync_tuser_1=off, c_s2mm_linebuffer_depth_1_sgadvanced=, c_s2mm_linebuffer_depth_1=0, c_s2mm_linebuffer_threshold_1=1, c_stream_if_configuration_2_sgadvanced=, c_stream_if_configuration_2=Master/Slave, c_no_of_frames_2=3, c_use_fsync_2_sgadvanced=, c_use_fsync_2=off, c_flush_on_fsync_2_sgadvanced=, c_flush_on_fsync_2=off, c_use_sg_engine_2_sgadvanced=, c_use_sg_engine_2=off, c_video_prm_read_2_sgadvanced=, c_video_prm_read_2=on, c_m_axis_mm2s_data_width_2_sgadvanced=, c_m_axis_mm2s_data_width_2=32, c_m_axis_mm2s_frame_sync_tuser_2_sgadvanced=, c_m_axis_mm2s_frame_sync_tuser_2=off, c_mm2s_linebuffer_depth_2_sgadvanced=, c_mm2s_linebuffer_depth_2=0, c_mm2s_linebuffer_threshold_2=1, c_s_axis_s2mm_data_width_2_sgadvanced=, c_s_axis_s2mm_data_width_2=32, c_s_axis_s2mm_frame_sync_tuser_2_sgadvanced=, c_s_axis_s2mm_frame_sync_tuser_2=off, c_s2mm_linebuffer_depth_2_sgadvanced=, c_s2mm_linebuffer_depth_2=0, c_s2mm_linebuffer_threshold_2=1, c_stream_if_configuration_3_sgadvanced=, c_stream_if_configuration_3=Master/Slave, c_no_of_frames_3=3, c_use_fsync_3_sgadvanced=, c_use_fsync_3=off, c_flush_on_fsync_3_sgadvanced=, c_flush_on_fsync_3=off, c_use_sg_engine_3_sgadvanced=, c_use_sg_engine_3=off, c_video_prm_read_3_sgadvanced=, c_video_prm_read_3=on, c_m_axis_mm2s_data_width_3_sgadvanced=, c_m_axis_mm2s_data_width_3=32, c_m_axis_mm2s_frame_sync_tuser_3_sgadvanced=, c_m_axis_mm2s_frame_sync_tuser_3=off, c_mm2s_linebuffer_depth_3_sgadvanced=, c_mm2s_linebuffer_depth_3=0, c_mm2s_linebuffer_threshold_3=1, c_s_axis_s2mm_data_width_3_sgadvanced=, c_s_axis_s2mm_data_width_3=32, c_s_axis_s2mm_frame_sync_tuser_3_sgadvanced=, c_s_axis_s2mm_frame_sync_tuser_3=off, c_s2mm_linebuffer_depth_3_sgadvanced=, c_s2mm_linebuffer_depth_3=0, c_s2mm_linebuffer_threshold_3=1, c_stream_if_configuration_4_sgadvanced=, c_stream_if_configuration_4=Master/Slave, c_no_of_frames_4=3, c_use_fsync_4_sgadvanced=, c_use_fsync_4=off, c_flush_on_fsync_4_sgadvanced=, c_flush_on_fsync_4=off, c_use_sg_engine_4_sgadvanced=, c_use_sg_engine_4=off, c_video_prm_read_4_sgadvanced=, c_video_prm_read_4=on, c_m_axis_mm2s_data_width_4_sgadvanced=, c_m_axis_mm2s_data_width_4=32, c_m_axis_mm2s_frame_sync_tuser_4_sgadvanced=, c_m_axis_mm2s_frame_sync_tuser_4=off, c_mm2s_linebuffer_depth_4_sgadvanced=, c_mm2s_linebuffer_depth_4=0, c_mm2s_linebuffer_threshold_4=1, c_s_axis_s2mm_data_width_4_sgadvanced=, c_s_axis_s2mm_data_width_4=32, c_s_axis_s2mm_frame_sync_tuser_4_sgadvanced=, c_s_axis_s2mm_frame_sync_tuser_4=off, c_s2mm_linebuffer_depth_4_sgadvanced=, c_s2mm_linebuffer_depth_4=0, c_s2mm_linebuffer_threshold_4=1, simulation_model='emi_v5_0:EMI_v5_0_Model', has_advanced_control=0, sggui_pos=-1,-1,-1,-1, block_type=vdma, block_version=, sg_icon_stat=335,743,15,20,white,yellow,0,c94a9c3c,right,,[2 2 2 2 2 2 2 2 3 3 3 3 3 4 1 ],[2 2 2 2 2 2 2 2 3 4 4 4 4 4 1 1 1 1 1 1 ], sg_mask_display=|, sg_list_contents=, sg_blockgui_xml=}
      mask sg_mask_display=|
      | fprintf('','COMMENT: begin icon graphics');
      | patch([0 0 5 5 ],[736 352 352 736 ],[7.375000e-001 7.225000e-001 5.125000e-001 ]);
      | patch([0 0 5 5 ],[336 102 102 336 ],[5.250000e-001 5.150000e-001 3.750000e-001 ]);
      | patch([0 0 5 5 ],[86 52 52 86 ],[3.125000e-001 3.075000e-001 2.375000e-001 ]);
      | patch([0 0 5 5 ],[36 2 2 36 ],[9.500000e-001 9.300000e-001 6.500000e-001 ]);
      | patch([330 330 335 335 ],[716 447 447 716 ],[7.375000e-001 7.225000e-001 5.125000e-001 ]);
      | patch([330 330 335 335 ],[436 412 412 436 ],[5.250000e-001 5.150000e-001 3.750000e-001 ]);
      | patch([330 330 335 335 ],[401 237 237 401 ],[3.125000e-001 3.075000e-001 2.375000e-001 ]);
      | patch([330 330 335 335 ],[226 27 27 226 ],[9.500000e-001 9.300000e-001 6.500000e-001 ]);
      | patch([5 329 329 5 5 ],[0 0 743 743 0 ],[9.500000e-001 9.300000e-001 6.500000e-001 ]);
      | plot([5 329 329 5 5 ],[0 0 743 743 0 ]);
      |
      |
      | patch([62.425 130.34 177.34 224.34 271.34 177.34 109.425 62.425 ],[423.17 423.17 470.17 423.17 470.17 470.17 470.17 423.17 ],[1 1 1 ]);
      | patch([109.425 177.34 130.34 62.425 109.425 ],[376.17 376.17 423.17 423.17 376.17 ],[0.985 0.979 0.895 ]);
      | patch([62.425 130.34 177.34 109.425 62.425 ],[329.17 329.17 376.17 376.17 329.17 ],[1 1 1 ]);
      | patch([109.425 271.34 224.34 177.34 130.34 62.425 109.425 ],[282.17 282.17 329.17 282.17 329.17 329.17 282.17 ],[0.985 0.979 0.895 ]);
      | fprintf('','COMMENT: end icon graphics');
      | fprintf('','COMMENT: begin icon text');
      | color('black');port_label('input',1,'  vdma_1_s_axi_lite_awvalid  ');
      | color('black');port_label('input',2,'  vdma_1_s_axi_lite_awaddr  ');
      | color('black');port_label('input',3,'  vdma_1_s_axi_lite_wvalid  ');
      | color('black');port_label('input',4,'  vdma_1_s_axi_lite_wdata  ');
      | color('black');port_label('input',5,'  vdma_1_s_axi_lite_bready  ');
      | color('black');port_label('input',6,'  vdma_1_s_axi_lite_arvalid  ');
      | color('black');port_label('input',7,'  vdma_1_s_axi_lite_araddr  ');
      | color('black');port_label('input',8,'  vdma_1_s_axi_lite_rready  ');
      | color('black');port_label('input',9,'  vdma_1_s_axis_s2mm_tdata  ');
      | color('black');port_label('input',10,'  vdma_1_s_axis_s2mm_tkeep  ');
      | color('black');port_label('input',11,'  vdma_1_s_axis_s2mm_tvalid  ');
      | color('black');port_label('input',12,'  vdma_1_s_axis_s2mm_tuser  ');
      | color('black');port_label('input',13,'  vdma_1_s_axis_s2mm_tlast  ');
      | color('black');port_label('input',14,'  vdma_1_m_axis_mm2s_tready  ');
      | color('black');port_label('input',15,'  vdma_1_axi_resetn  ');
      | color('black');port_label('output',1,'  vdma_1_s_axi_lite_awready  ');
      | color('black');port_label('output',2,'  vdma_1_s_axi_lite_wready  ');
      | color('black');port_label('output',3,'  vdma_1_s_axi_lite_bresp  ');
      | color('black');port_label('output',4,'  vdma_1_s_axi_lite_bvalid  ');
      | color('black');port_label('output',5,'  vdma_1_s_axi_lite_arready  ');
      | color('black');port_label('output',6,'  vdma_1_s_axi_lite_rvalid  ');
      | color('black');port_label('output',7,'  vdma_1_s_axi_lite_rdata  ');
      | color('black');port_label('output',8,'  vdma_1_s_axi_lite_rresp  ');
      | color('black');port_label('output',9,'  vdma_1_s_axis_s2mm_tready  ');
      | color('black');port_label('output',10,'  vdma_1_m_axis_mm2s_tdata  ');
      | color('black');port_label('output',11,'  vdma_1_m_axis_mm2s_tkeep  ');
      | color('black');port_label('output',12,'  vdma_1_m_axis_mm2s_tvalid  ');
      | color('black');port_label('output',13,'  vdma_1_m_axis_mm2s_tuser  ');
      | color('black');port_label('output',14,'  vdma_1_m_axis_mm2s_tlast  ');
      | color('black');port_label('output',15,'  vdma_1_mm2s_introut  ');
      | color('black');port_label('output',16,'  vdma_1_mm2s_fsync_out  ');
      | color('black');port_label('output',17,'  vdma_1_mm2s_prmtr_update  ');
      | color('black');port_label('output',18,'  vdma_1_s2mm_introut  ');
      | color('black');port_label('output',19,'  vdma_1_s2mm_fsync_out  ');
      | color('black');port_label('output',20,'  vdma_1_s2mm_prmtr_update  ');
      | fprintf('','COMMENT: end icon text');
      mask prompts: infoedit ""; c_mem_size_sgadvanced ""; c_mem_size "Memory size"; c_number_of_vdma_if_sgadvanced ""; c_number_of_vdma_if "Number of VDMA interfaces"; c_stream_if_configuration_1_sgadvanced ""; c_stream_if_configuration_1 "Stream interface"; c_no_of_frames_1 "Number of frame stores [1..32]"; c_use_fsync_1_sgadvanced ""; c_use_fsync_1 "Use external frame sync"; c_flush_on_fsync_1_sgadvanced ""; c_flush_on_fsync_1 "Flush on frame sync"; c_use_sg_engine_1_sgadvanced ""; c_use_sg_engine_1 "Use Scatter Gather Engine"; c_video_prm_read_1_sgadvanced ""; c_video_prm_read_1 "Use Video Parameter Read for Direct Mode"; c_m_axis_mm2s_data_width_1_sgadvanced ""; c_m_axis_mm2s_data_width_1 "Data width"; c_m_axis_mm2s_frame_sync_tuser_1_sgadvanced ""; c_m_axis_mm2s_frame_sync_tuser_1 "Frame sync on TUSER(0)"; c_mm2s_linebuffer_depth_1_sgadvanced ""; c_mm2s_linebuffer_depth_1 "Depth"; c_mm2s_linebuffer_threshold_1 "Almost empty threshold [1..65536]"; c_s_axis_s2mm_data_width_1_sgadvanced ""; c_s_axis_s2mm_data_width_1 "Data width"; c_s_axis_s2mm_frame_sync_tuser_1_sgadvanced ""; c_s_axis_s2mm_frame_sync_tuser_1 "Frame sync on TUSER(0)"; c_s2mm_linebuffer_depth_1_sgadvanced ""; c_s2mm_linebuffer_depth_1 "Depth"; c_s2mm_linebuffer_threshold_1 "Almost full threshold [1..65536]"; c_stream_if_configuration_2_sgadvanced ""; c_stream_if_configuration_2 "Stream interface"; c_no_of_frames_2 "Number of frame stores [1..32]"; c_use_fsync_2_sgadvanced ""; c_use_fsync_2 "Use external frame sync"; c_flush_on_fsync_2_sgadvanced ""; c_flush_on_fsync_2 "Flush on frame sync"; c_use_sg_engine_2_sgadvanced ""; c_use_sg_engine_2 "Use Scatter Gather Engine"; c_video_prm_read_2_sgadvanced ""; c_video_prm_read_2 "Use Video Parameter Read for Direct Mode"; c_m_axis_mm2s_data_width_2_sgadvanced ""; c_m_axis_mm2s_data_width_2 "Data width"; c_m_axis_mm2s_frame_sync_tuser_2_sgadvanced ""; c_m_axis_mm2s_frame_sync_tuser_2 "Frame sync on TUSER(0)"; c_mm2s_linebuffer_depth_2_sgadvanced ""; c_mm2s_linebuffer_depth_2 "Depth"; c_mm2s_linebuffer_threshold_2 "Almost empty threshold [1..65536]"; c_s_axis_s2mm_data_width_2_sgadvanced ""; c_s_axis_s2mm_data_width_2 "Data width"; c_s_axis_s2mm_frame_sync_tuser_2_sgadvanced ""; c_s_axis_s2mm_frame_sync_tuser_2 "Frame sync on TUSER(0)"; c_s2mm_linebuffer_depth_2_sgadvanced ""; c_s2mm_linebuffer_depth_2 "Depth"; c_s2mm_linebuffer_threshold_2 "Almost full threshold [1..65536]"; c_stream_if_configuration_3_sgadvanced ""; c_stream_if_configuration_3 "Stream interface"; c_no_of_frames_3 "Number of frame stores [1..32]"; c_use_fsync_3_sgadvanced ""; c_use_fsync_3 "Use external frame sync"; c_flush_on_fsync_3_sgadvanced ""; c_flush_on_fsync_3 "Flush on frame sync"; c_use_sg_engine_3_sgadvanced ""; c_use_sg_engine_3 "Use Scatter Gather Engine"; c_video_prm_read_3_sgadvanced ""; c_video_prm_read_3 "Use Video Parameter Read for Direct Mode"; c_m_axis_mm2s_data_width_3_sgadvanced ""; c_m_axis_mm2s_data_width_3 "Data width"; c_m_axis_mm2s_frame_sync_tuser_3_sgadvanced ""; c_m_axis_mm2s_frame_sync_tuser_3 "Frame sync on TUSER(0)"; c_mm2s_linebuffer_depth_3_sgadvanced ""; c_mm2s_linebuffer_depth_3 "Depth"; c_mm2s_linebuffer_threshold_3 "Almost empty threshold [1..65536]"; c_s_axis_s2mm_data_width_3_sgadvanced ""; c_s_axis_s2mm_data_width_3 "Data width"; c_s_axis_s2mm_frame_sync_tuser_3_sgadvanced ""; c_s_axis_s2mm_frame_sync_tuser_3 "Frame sync on TUSER(0)"; c_s2mm_linebuffer_depth_3_sgadvanced ""; c_s2mm_linebuffer_depth_3 "Depth"; c_s2mm_linebuffer_threshold_3 "Almost full threshold [1..65536]"; c_stream_if_configuration_4_sgadvanced ""; c_stream_if_configuration_4 "Stream interface"; c_no_of_frames_4 "Number of frame stores [1..32]"; c_use_fsync_4_sgadvanced ""; c_use_fsync_4 "Use external frame sync"; c_flush_on_fsync_4_sgadvanced ""; c_flush_on_fsync_4 "Flush on frame sync"; c_use_sg_engine_4_sgadvanced ""; c_use_sg_engine_4 "Use Scatter Gather Engine"; c_video_prm_read_4_sgadvanced ""; c_video_prm_read_4 "Use Video Parameter Read for Direct Mode"; c_m_axis_mm2s_data_width_4_sgadvanced ""; c_m_axis_mm2s_data_width_4 "Data width"; c_m_axis_mm2s_frame_sync_tuser_4_sgadvanced ""; c_m_axis_mm2s_frame_sync_tuser_4 "Frame sync on TUSER(0)"; c_mm2s_linebuffer_depth_4_sgadvanced ""; c_mm2s_linebuffer_depth_4 "Depth"; c_mm2s_linebuffer_threshold_4 "Almost empty threshold [1..65536]"; c_s_axis_s2mm_data_width_4_sgadvanced ""; c_s_axis_s2mm_data_width_4 "Data width"; c_s_axis_s2mm_frame_sync_tuser_4_sgadvanced ""; c_s_axis_s2mm_frame_sync_tuser_4 "Frame sync on TUSER(0)"; c_s2mm_linebuffer_depth_4_sgadvanced ""; c_s2mm_linebuffer_depth_4 "Depth"; c_s2mm_linebuffer_threshold_4 "Almost full threshold [1..65536]"; simulation_model ""; has_advanced_control ""; sggui_pos ""; block_type ""; block_version ""; sg_icon_stat ""; sg_mask_display ""; sg_list_contents ""; sg_blockgui_xml ""
      mask help: This is a bit-accurate simulation model for multiple AXI VDMA external memory interfaces. Netlisting will generate the port interface that can be attached to the VDMA IP. This block is currently in beta.
      mask init:
      | try
      |   tmp_gcb = gcb;
      |   tmp_gcbh = gcbh;
      |   if (strcmp('SysGenIndex',get_param(bdroot(tmp_gcbh),'tag')) && ~isempty(regexp(bdroot(tmp_gcb), '^xbs', 'once')))
      |     return;
      |   end;
      |   xlMungeMaskParams;
      |   block_config = 'emi_v5_0:emi_all_interfaces_config';
      | 
      |   block_type='vdma';
      | 
      |   serialized_declarations = '{''c_flush_on_fsync_1''=>''Int'',''c_flush_on_fsync_2''=>''Int'',''c_flush_on_fsync_3''=>''Int'',''c_flush_on_fsync_4''=>''Int'',''c_m_axis_mm2s_data_width_1''=>''Int'',''c_m_axis_mm2s_data_width_2''=>''Int'',''c_m_axis_mm2s_data_width_3''=>''Int'',''c_m_axis_mm2s_data_width_4''=>''Int'',''c_m_axis_mm2s_frame_sync_tuser_1''=>''Int'',''c_m_axis_mm2s_frame_sync_tuser_2''=>''Int'',''c_m_axis_mm2s_frame_sync_tuser_3''=>''Int'',''c_m_axis_mm2s_frame_sync_tuser_4''=>''Int'',''c_mem_size''=>''Int'',''c_mm2s_linebuffer_depth_1''=>''Int'',''c_mm2s_linebuffer_depth_2''=>''Int'',''c_mm2s_linebuffer_depth_3''=>''Int'',''c_mm2s_linebuffer_depth_4''=>''Int'',''c_mm2s_linebuffer_threshold_1''=>''Int'',''c_mm2s_linebuffer_threshold_2''=>''Int'',''c_mm2s_linebuffer_threshold_3''=>''Int'',''c_mm2s_linebuffer_threshold_4''=>''Int'',''c_no_of_frames_1''=>''Int'',''c_no_of_frames_2''=>''Int'',''c_no_of_frames_3''=>''Int'',''c_no_of_frames_4''=>''Int'',''c_number_of_vdma_if''=>''Int'',''c_s2mm_linebuffer_depth_1''=>''Int'',''c_s2mm_linebuffer_depth_2''=>''Int'',''c_s2mm_linebuffer_depth_3''=>''Int'',''c_s2mm_linebuffer_depth_4''=>''Int'',''c_s2mm_linebuffer_threshold_1''=>''Int'',''c_s2mm_linebuffer_threshold_2''=>''Int'',''c_s2mm_linebuffer_threshold_3''=>''Int'',''c_s2mm_linebuffer_threshold_4''=>''Int'',''c_s_axis_s2mm_data_width_1''=>''Int'',''c_s_axis_s2mm_data_width_2''=>''Int'',''c_s_axis_s2mm_data_width_3''=>''Int'',''c_s_axis_s2mm_data_width_4''=>''Int'',''c_s_axis_s2mm_frame_sync_tuser_1''=>''Int'',''c_s_axis_s2mm_frame_sync_tuser_2''=>''Int'',''c_s_axis_s2mm_frame_sync_tuser_3''=>''Int'',''c_s_axis_s2mm_frame_sync_tuser_4''=>''Int'',''c_stream_if_configuration_1''=>''Int'',''c_stream_if_configuration_2''=>''Int'',''c_stream_if_configuration_3''=>''Int'',''c_stream_if_configuration_4''=>''Int'',''c_use_fsync_1''=>''Int'',''c_use_fsync_2''=>''Int'',''c_use_fsync_3''=>''Int'',''c_use_fsync_4''=>''Int'',''c_use_sg_engine_1''=>''Int'',''c_use_sg_engine_2''=>''Int'',''c_use_sg_engine_3''=>''Int'',''c_use_sg_engine_4''=>''Int'',''c_video_prm_read_1''=>''Int'',''c_video_prm_read_2''=>''Int'',''c_video_prm_read_3''=>''Int'',''c_video_prm_read_4''=>''Int'',''simulation_model''=>''String'',''block_type''=>''String''}';
      |   ptable_ = xlblockprep(get_param(tmp_gcb, 'MaskWSVariables'));
      |   try
      |     xlBlockMoveCallback(tmp_gcbh);
      |   catch 
      |      clear global xl_updateicon_recursion_guard;
      |   end;
      | catch
      |   global dbgsysgen;
      |   if(~isempty(dbgsysgen) && dbgsysgen)
      |     e = regexprep(lasterr, '\n', '\nError: ');
      |     disp(['Error: While running MaskInit code on block ' tmp_gcb ': ' e]);
      |     error(e);
      |   end
      | end
      settings: CopyFcn=xlBlockMoveCallback(gcbh);  DeleteFcn=xlDestroyGui(gcbh);  ModelCloseFcn=xlDestroyGui(gcbh);  PreSaveFcn=xlBlockPreSaveCallback(gcbh);  PostSaveFcn=xlBlockPostSaveCallback(gcbh);  DestroyFcn=xlDestroyGui(gcbh);  OpenFcn=xlOpenGui(gcbh, 'vdma_v5_0_gui.xml', @xlEMIEnablement_v5_0, @xlEMIaction_v5_0)  CloseFcn=xlDestroyGui(gcbh);  MoveFcn=xlBlockMoveCallback(gcbh);
      mask Help: eval('');xlDoc('-book','sysgen','-topic','VDMA_Interface_5_0');
      mask StyleString: edit,edit,popup(16MB|32MB|64MB|128MB|256MB|512MB|1GB|2GB),edit,popup(1|2|3|4),edit,popup(Master/Slave|Master|Slave),edit,edit,checkbox,edit,checkbox,edit,checkbox,edit,checkbox,edit,popup(8|16|32|64|128|256|512|1024),edit,checkbox,edit,popup(0|1|2|4|8|16|32|64|128|256|512|1024|2048|4096|8192|16384|32768|65536),edit,edit,popup(8|16|32|64|128|256|512|1024),edit,checkbox,edit,popup(0|1|2|4|8|16|32|64|128|256|512|1024|2048|4096|8192|16384|32768|65536),edit,edit,popup(Master/Slave|Master|Slave),edit,edit,checkbox,edit,checkbox,edit,checkbox,edit,checkbox,edit,popup(8|16|32|64|128|256|512|1024),edit,checkbox,edit,popup(0|1|2|4|8|16|32|64|128|256|512|1024|2048|4096|8192|16384|32768|65536),edit,edit,popup(8|16|32|64|128|256|512|1024),edit,checkbox,edit,popup(0|1|2|4|8|16|32|64|128|256|512|1024|2048|4096|8192|16384|32768|65536),edit,edit,popup(Master/Slave|Master|Slave),edit,edit,checkbox,edit,checkbox,edit,checkbox,edit,checkbox,edit,popup(8|16|32|64|128|256|512|1024),edit,checkbox,edit,popup(0|1|2|4|8|16|32|64|128|256|512|1024|2048|4096|8192|16384|32768|65536),edit,edit,popup(8|16|32|64|128|256|512|1024),edit,checkbox,edit,popup(0|1|2|4|8|16|32|64|128|256|512|1024|2048|4096|8192|16384|32768|65536),edit,edit,popup(Master/Slave|Master|Slave),edit,edit,checkbox,edit,checkbox,edit,checkbox,edit,checkbox,edit,popup(8|16|32|64|128|256|512|1024),edit,checkbox,edit,popup(0|1|2|4|8|16|32|64|128|256|512|1024|2048|4096|8192|16384|32768|65536),edit,edit,popup(8|16|32|64|128|256|512|1024),edit,checkbox,edit,popup(0|1|2|4|8|16|32|64|128|256|512|1024|2048|4096|8192|16384|32768|65536),edit,edit,edit,edit,edit,edit,edit,edit,edit,edit
      mask Display:
      | fprintf('','COMMENT: begin icon graphics');
      | patch([0 0 5 5 ],[736 352 352 736 ],[7.375000e-001 7.225000e-001 5.125000e-001 ]);
      | patch([0 0 5 5 ],[336 102 102 336 ],[5.250000e-001 5.150000e-001 3.750000e-001 ]);
      | patch([0 0 5 5 ],[86 52 52 86 ],[3.125000e-001 3.075000e-001 2.375000e-001 ]);
      | patch([0 0 5 5 ],[36 2 2 36 ],[9.500000e-001 9.300000e-001 6.500000e-001 ]);
      | patch([330 330 335 335 ],[716 447 447 716 ],[7.375000e-001 7.225000e-001 5.125000e-001 ]);
      | patch([330 330 335 335 ],[436 412 412 436 ],[5.250000e-001 5.150000e-001 3.750000e-001 ]);
      | patch([330 330 335 335 ],[401 237 237 401 ],[3.125000e-001 3.075000e-001 2.375000e-001 ]);
      | patch([330 330 335 335 ],[226 27 27 226 ],[9.500000e-001 9.300000e-001 6.500000e-001 ]);
      | patch([5 329 329 5 5 ],[0 0 743 743 0 ],[9.500000e-001 9.300000e-001 6.500000e-001 ]);
      | plot([5 329 329 5 5 ],[0 0 743 743 0 ]);
      | 
      | 
      | patch([62.425 130.34 177.34 224.34 271.34 177.34 109.425 62.425 ],[423.17 423.17 470.17 423.17 470.17 470.17 470.17 423.17 ],[1 1 1 ]);
      | patch([109.425 177.34 130.34 62.425 109.425 ],[376.17 376.17 423.17 423.17 376.17 ],[0.985 0.979 0.895 ]);
      | patch([62.425 130.34 177.34 109.425 62.425 ],[329.17 329.17 376.17 376.17 329.17 ],[1 1 1 ]);
      | patch([109.425 271.34 224.34 177.34 130.34 62.425 109.425 ],[282.17 282.17 329.17 282.17 329.17 329.17 282.17 ],[0.985 0.979 0.895 ]);
      | fprintf('','COMMENT: end icon graphics');
      | fprintf('','COMMENT: begin icon text');
      | color('black');port_label('input',1,'  vdma_1_s_axi_lite_awvalid  ');
      | color('black');port_label('input',2,'  vdma_1_s_axi_lite_awaddr  ');
      | color('black');port_label('input',3,'  vdma_1_s_axi_lite_wvalid  ');
      | color('black');port_label('input',4,'  vdma_1_s_axi_lite_wdata  ');
      | color('black');port_label('input',5,'  vdma_1_s_axi_lite_bready  ');
      | color('black');port_label('input',6,'  vdma_1_s_axi_lite_arvalid  ');
      | color('black');port_label('input',7,'  vdma_1_s_axi_lite_araddr  ');
      | color('black');port_label('input',8,'  vdma_1_s_axi_lite_rready  ');
      | color('black');port_label('input',9,'  vdma_1_s_axis_s2mm_tdata  ');
      | color('black');port_label('input',10,'  vdma_1_s_axis_s2mm_tkeep  ');
      | color('black');port_label('input',11,'  vdma_1_s_axis_s2mm_tvalid  ');
      | color('black');port_label('input',12,'  vdma_1_s_axis_s2mm_tuser  ');
      | color('black');port_label('input',13,'  vdma_1_s_axis_s2mm_tlast  ');
      | color('black');port_label('input',14,'  vdma_1_m_axis_mm2s_tready  ');
      | color('black');port_label('input',15,'  vdma_1_axi_resetn  ');
      | color('black');port_label('output',1,'  vdma_1_s_axi_lite_awready  ');
      | color('black');port_label('output',2,'  vdma_1_s_axi_lite_wready  ');
      | color('black');port_label('output',3,'  vdma_1_s_axi_lite_bresp  ');
      | color('black');port_label('output',4,'  vdma_1_s_axi_lite_bvalid  ');
      | color('black');port_label('output',5,'  vdma_1_s_axi_lite_arready  ');
      | color('black');port_label('output',6,'  vdma_1_s_axi_lite_rvalid  ');
      | color('black');port_label('output',7,'  vdma_1_s_axi_lite_rdata  ');
      | color('black');port_label('output',8,'  vdma_1_s_axi_lite_rresp  ');
      | color('black');port_label('output',9,'  vdma_1_s_axis_s2mm_tready  ');
      | color('black');port_label('output',10,'  vdma_1_m_axis_mm2s_tdata  ');
      | color('black');port_label('output',11,'  vdma_1_m_axis_mm2s_tkeep  ');
      | color('black');port_label('output',12,'  vdma_1_m_axis_mm2s_tvalid  ');
      | color('black');port_label('output',13,'  vdma_1_m_axis_mm2s_tuser  ');
      | color('black');port_label('output',14,'  vdma_1_m_axis_mm2s_tlast  ');
      | color('black');port_label('output',15,'  vdma_1_mm2s_introut  ');
      | color('black');port_label('output',16,'  vdma_1_mm2s_fsync_out  ');
      | color('black');port_label('output',17,'  vdma_1_mm2s_prmtr_update  ');
      | color('black');port_label('output',18,'  vdma_1_s2mm_introut  ');
      | color('black');port_label('output',19,'  vdma_1_s2mm_fsync_out  ');
      | color('black');port_label('output',20,'  vdma_1_s2mm_prmtr_update  ');
      | fprintf('','COMMENT: end icon text');
  "Viterbi Decoder 7.0 " : S-Function  LoadFcn=xlBlockLoadCallback(gcbh);  FunctionName=sysgen  Parameters=ptable_  EnableBusSupport=off  mask(Xilinx Viterbi Decoder 7.0  Block){channels=1, viterbi_type_sgadvanced=, viterbi_type=Standard, reduced_latency_sgadvanced=, reduced_latency=off, constraint_length=7, traceback_length=42, architecture_sgadvanced=, architecture=Parallel, best_state_sgadvanced=, best_state=on, best_state_width=3, soft_width=3, coding_sgadvanced=, coding=Soft_Coding, data_format_sgadvanced=, data_format=Signed_Magnitude, output_rate0=2, convolution_code_0_radix=Binary, convolution0_code0='1111001', convolution0_code1='1011011', convolution0_code2='0', convolution0_code3='0', convolution0_code4='0', convolution0_code5='0', convolution0_code6='0', output_rate1=2, convolution_code_1_radix=Binary, convolution1_code0='1111001', convolution1_code1='1011011', convolution1_code2='0', convolution1_code3='0', convolution1_code4='0', convolution1_code5='0', convolution1_code6='0', trellis_initialization_sgadvanced=, trellis_initialization=None, maximum_direct=42, direct_traceback_sgadvanced=, direct_traceback=None, puncturing_sgadvanced=, puncturing=None, ber_symbol_count_sgadvanced=, ber_symbol_count=on, number_of_ber_symbols=300, synchronization_sgadvanced=, synchronization=off, dynamic_thresholds_sgadvanced=, dynamic_thresholds=off, ber_thresh=600, norm_thresh=250, ce_sgadvanced=, ce=off, rdy_sgadvanced=, rdy=off, synchronous_clear_sgadvanced=, synchronous_clear=off, norm_sgadvanced=, norm=off, block_valid_sgadvanced=, block_valid=off, ip_name=Viterbi Decoder, ip_version=7.0, dsptool_ready=false, ipcore_usecache=true, ipcore_useipmodelcache=true, wrapper_available=true, port_translation_map={ 'ce' => 'en', 'sclr' => 'rst'}, structural_sim=false, has_advanced_control=0, sggui_pos=-1,-1,-1,-1, block_type=viterbi_v7_0, block_version=, sg_icon_stat=95,142,2,3,white,green,0,d403ebf9,right,,[ ],[ ], sg_mask_display=|, sg_list_contents=, sg_blockgui_xml=}
      mask sg_mask_display=|
      | fprintf('','COMMENT: begin icon graphics');
      | patch([0 95 95 0 0 ],[0 0 142 142 0 ],[0.72 0.84 0.7 ]);
      | plot([0 95 95 0 0 ],[0 0 142 142 0 ]);
      | patch([18.075 36.86 49.86 62.86 75.86 49.86 31.075 18.075 ],[85.43 85.43 98.43 85.43 98.43 98.43 98.43 85.43 ],[1 1 1 ]);
      | patch([31.075 49.86 36.86 18.075 31.075 ],[72.43 72.43 85.43 85.43 72.43 ],[0.916 0.952 0.91 ]);
      | patch([18.075 36.86 49.86 31.075 18.075 ],[59.43 59.43 72.43 72.43 59.43 ],[1 1 1 ]);
      | patch([31.075 75.86 62.86 49.86 36.86 18.075 31.075 ],[46.43 46.43 59.43 46.43 59.43 59.43 46.43 ],[0.916 0.952 0.91 ]);
      | fprintf('','COMMENT: end icon graphics');
      | fprintf('','COMMENT: begin icon text');
      | color('black');port_label('input',1,'data_in0');
      | color('black');port_label('input',2,'data_in1');
      | color('black');port_label('output',1,'data_out');
      | color('black');port_label('output',2,'ber');
      | color('black');port_label('output',3,'ber_done');
      | fprintf('','COMMENT: end icon text');
      mask prompts: channels "Number of Channels"; viterbi_type_sgadvanced ""; viterbi_type ""; reduced_latency_sgadvanced ""; reduced_latency "Use Reduced Latency"; constraint_length "Constraint Length"; traceback_length "Traceback Length"; architecture_sgadvanced ""; architecture ""; best_state_sgadvanced ""; best_state "Use Best State"; best_state_width "Best State Width"; soft_width "Soft Width"; coding_sgadvanced ""; coding ""; data_format_sgadvanced ""; data_format ""; output_rate0 "Output Rate 0"; convolution_code_0_radix "Convolution Code 0 Radix"; convolution0_code0 "Convolution 0 Code 0"; convolution0_code1 "Convolution 0 Code 1"; convolution0_code2 "Convolution 0 Code 2"; convolution0_code3 "Convolution 0 Code 3"; convolution0_code4 "Convolution 0 Code 4"; convolution0_code5 "Convolution 0 Code 5"; convolution0_code6 "Convolution 0 Code 6"; output_rate1 "Output Rate 1"; convolution_code_1_radix "Convolution Code 1 Radix"; convolution1_code0 "Convolution 1 Code 0"; convolution1_code1 "Convolution 1 Code 1"; convolution1_code2 "Convolution 1 Code 2"; convolution1_code3 "Convolution 1 Code 3"; convolution1_code4 "Convolution 1 Code 4"; convolution1_code5 "Convolution 1 Code 5"; convolution1_code6 "Convolution 1 Code 6"; trellis_initialization_sgadvanced ""; trellis_initialization ""; maximum_direct "Maximum Direct"; direct_traceback_sgadvanced ""; direct_traceback ""; puncturing_sgadvanced ""; puncturing ""; ber_symbol_count_sgadvanced ""; ber_symbol_count "Use BER Symbol Count"; number_of_ber_symbols "Number of BER Symbols"; synchronization_sgadvanced ""; synchronization "Use Synchronization"; dynamic_thresholds_sgadvanced ""; dynamic_thresholds "Use Dynamic Thresholds"; ber_thresh "BER Thresh"; norm_thresh "Norm Thresh"; ce_sgadvanced ""; rdy_sgadvanced ""; synchronous_clear_sgadvanced ""; synchronous_clear "SCLR"; norm_sgadvanced ""; block_valid_sgadvanced ""; block_valid "Block Valid"; ip_name ""; ip_version ""; dsptool_ready ""; ipcore_usecache ""; ipcore_useipmodelcache ""; wrapper_available ""; port_translation_map ""; structural_sim ""; has_advanced_control ""; sggui_pos ""; block_type ""; block_version ""; sg_icon_stat ""; sg_mask_display ""; sg_list_contents ""; sg_blockgui_xml ""
      mask help: Xilinx Viterbi Decoder 7.0
      mask init:
      | try
      |   tmp_gcb = gcb;
      |   tmp_gcbh = gcbh;
      |   if (strcmp('SysGenIndex',get_param(bdroot(tmp_gcbh),'tag')) && ~isempty(regexp(bdroot(tmp_gcb), '^xbs', 'once')))
      |     return;
      |   end;
      |   xlMungeMaskParams;
      |   block_config = 'sysgen:coregenimport_config';
      | 
      |   block_type='viterbi_v7_0';
      | 
      |   serialized_declarations = '{''architecture''=>''String'',''ber_symbol_count''=>''Bool'',''ber_thresh''=>''Int'',''best_state''=>''Bool'',''best_state_width''=>''Int'',''block_valid''=>''Bool'',''ce''=>''Bool'',''channels''=>''Int'',''coding''=>''String'',''constraint_length''=>''Int'',''convolution0_code0''=>''String'',''convolution0_code1''=>''String'',''convolution0_code2''=>''String'',''convolution0_code3''=>''String'',''convolution0_code4''=>''String'',''convolution0_code5''=>''String'',''convolution0_code6''=>''String'',''convolution1_code0''=>''String'',''convolution1_code1''=>''String'',''convolution1_code2''=>''String'',''convolution1_code3''=>''String'',''convolution1_code4''=>''String'',''convolution1_code5''=>''String'',''convolution1_code6''=>''String'',''convolution_code_0_radix''=>''String'',''convolution_code_1_radix''=>''String'',''data_format''=>''String'',''direct_traceback''=>''String'',''dsptool_ready''=>''Bool'',''dynamic_thresholds''=>''Bool'',''ip_name''=>''String'',''ip_version''=>''String'',''ipcore_usecache''=>''Bool'',''ipcore_useipmodelcache''=>''Bool'',''maximum_direct''=>''Int'',''norm''=>''Bool'',''norm_thresh''=>''Int'',''number_of_ber_symbols''=>''Int'',''output_rate0''=>''Int'',''output_rate1''=>''Int'',''port_translation_map''=>''String'',''puncturing''=>''String'',''rdy''=>''Bool'',''reduced_latency''=>''Bool'',''soft_width''=>''Int'',''structural_sim''=>''Bool'',''synchronization''=>''Bool'',''synchronous_clear''=>''Bool'',''traceback_length''=>''Int'',''trellis_initialization''=>''String'',''viterbi_type''=>''String'',''wrapper_available''=>''Bool'',''block_type''=>''String''}';
      |   ptable_ = xlblockprep(get_param(tmp_gcb, 'MaskWSVariables'));
      |   try
      |     xlBlockMoveCallback(tmp_gcbh);
      |   catch 
      |      clear global xl_updateicon_recursion_guard;
      |   end;
      | catch
      |   global dbgsysgen;
      |   if(~isempty(dbgsysgen) && dbgsysgen)
      |     e = regexprep(lasterr, '\n', '\nError: ');
      |     disp(['Error: While running MaskInit code on block ' tmp_gcb ': ' e]);
      |     error(e);
      |   end
      | end
      settings: CopyFcn=xlBlockMoveCallback(gcbh);  DeleteFcn=xlDestroyGui(gcbh);  ModelCloseFcn=xlDestroyGui(gcbh);  PreSaveFcn=xlBlockPreSaveCallback(gcbh);  PostSaveFcn=xlBlockPostSaveCallback(gcbh);  DestroyFcn=xlDestroyGui(gcbh);  OpenFcn=xlOpenGui(gcbh, 'viterbi_v7_0_gui.xml', @xlipmagiccallback_pass_evaluate_params, @xlipmagicaction)  CloseFcn=xlDestroyGui(gcbh);  MoveFcn=xlBlockMoveCallback(gcbh);
      mask Help: eval('');xlDoc('-book','sysgen','-topic','Viterbi_Decoder_7_0');
      mask StyleString: edit,edit,popup(Standard|Multi_Channel|Trellis_Mode|Dual_Decoder),edit,checkbox,edit,edit,edit,popup(Parallel|Serial),edit,checkbox,edit,edit,edit,popup(Soft_Coding|Hard_Coding),edit,popup(Signed_Magnitude|Offset_Binary),edit,popup(Binary|Octal|Decimal),edit,edit,edit,edit,edit,edit,edit,edit,popup(Binary|Octal|Decimal),edit,edit,edit,edit,edit,edit,edit,edit,popup(None|State_Zero|Equal_States|User_Input),edit,edit,popup(None|State_Zero|User_Input|Best_State),edit,popup(None|External),edit,checkbox,edit,edit,checkbox,edit,checkbox,edit,edit,edit,checkbox,edit,checkbox,edit,checkbox,edit,checkbox,edit,checkbox,edit,edit,edit,edit,edit,edit,edit,edit,edit,edit,edit,edit,edit,edit,edit,edit
      mask Display:
      | fprintf('','COMMENT: begin icon graphics');
      | patch([0 95 95 0 0 ],[0 0 142 142 0 ],[0.72 0.84 0.7 ]);
      | plot([0 95 95 0 0 ],[0 0 142 142 0 ]);
      | patch([18.075 36.86 49.86 62.86 75.86 49.86 31.075 18.075 ],[85.43 85.43 98.43 85.43 98.43 98.43 98.43 85.43 ],[1 1 1 ]);
      | patch([31.075 49.86 36.86 18.075 31.075 ],[72.43 72.43 85.43 85.43 72.43 ],[0.916 0.952 0.91 ]);
      | patch([18.075 36.86 49.86 31.075 18.075 ],[59.43 59.43 72.43 72.43 59.43 ],[1 1 1 ]);
      | patch([31.075 75.86 62.86 49.86 36.86 18.075 31.075 ],[46.43 46.43 59.43 46.43 59.43 59.43 46.43 ],[0.916 0.952 0.91 ]);
      | fprintf('','COMMENT: end icon graphics');
      | fprintf('','COMMENT: begin icon text');
      | color('black');port_label('input',1,'data_in0');
      | color('black');port_label('input',2,'data_in1');
      | color('black');port_label('output',1,'data_out');
      | color('black');port_label('output',2,'ber');
      | color('black');port_label('output',3,'ber_done');
      | fprintf('','COMMENT: end icon text');
  "Viterbi Decoder 8.0 " : S-Function  LoadFcn=xlBlockLoadCallback(gcbh);  FunctionName=sysgen  Parameters=ptable_  EnableBusSupport=off  mask(Xilinx Viterbi Decoder 8.0  Block){channels=1, viterbi_type_sgadvanced=, viterbi_type=Standard, reduced_latency_sgadvanced=, reduced_latency=off, constraint_length=7, traceback_length=42, architecture_sgadvanced=, architecture=Parallel, best_state_sgadvanced=, best_state=on, best_state_width=3, puncturing_sgadvanced=, puncturing=None, soft_width=3, coding_sgadvanced=, coding=Soft_Coding, data_format_sgadvanced=, data_format=Signed_Magnitude, output_rate0=2, convolution_code_0_radix=Binary, convolution0_code0='1111001', convolution0_code1='1011011', convolution0_code2='0', convolution0_code3='0', convolution0_code4='0', convolution0_code5='0', convolution0_code6='0', output_rate1=2, convolution_code_1_radix=Binary, convolution1_code0='1111001', convolution1_code1='1011011', convolution1_code2='0', convolution1_code3='0', convolution1_code4='0', convolution1_code5='0', convolution1_code6='0', ber_symbol_count_sgadvanced=, ber_symbol_count=on, norm_sgadvanced=, norm=off, block_valid_sgadvanced=, block_valid=off, tready_sgadvanced=, tready=on, aclken_sgadvanced=, aclken=off, aresetn_sgadvanced=, aresetn=off, trim_axipin_name=on, ip_name=Viterbi Decoder, ip_version=8.0, dsptool_ready=false, ipcore_usecache=true, ipcore_useipmodelcache=true, wrapper_available=true, port_translation_map={ 'aclken' => 'en', 'aresetn' => 'rst'}, structural_sim=false, has_advanced_control=0, sggui_pos=-1,-1,-1,-1, block_type=viterbi_v8_0, block_version=, sg_icon_stat=215,240,7,6,white,green,0,f50cc4d1,right,,[2 2 2 3 3 4 5 ],[2 3 4 4 5 5 ], sg_mask_display=|, sg_list_contents=, sg_blockgui_xml=}
      mask sg_mask_display=|
      | fprintf('','COMMENT: begin icon graphics');
      | patch([0 0 4 4 ],[237 143 143 237 ],[5.960000e-001 6.920000e-001 5.800000e-001 ]);
      | patch([0 0 4 4 ],[132 73 73 132 ],[4.720000e-001 5.440000e-001 4.600000e-001 ]);
      | patch([0 0 4 4 ],[62 38 38 62 ],[3.480000e-001 3.960000e-001 3.400000e-001 ]);
      | patch([0 0 4 4 ],[27 3 3 27 ],[2.240000e-001 2.480000e-001 2.200000e-001 ]);
      | patch([211 211 215 215 ],[234 206 206 234 ],[5.960000e-001 6.920000e-001 5.800000e-001 ]);
      | patch([211 211 215 215 ],[194 166 166 194 ],[4.720000e-001 5.440000e-001 4.600000e-001 ]);
      | patch([211 211 215 215 ],[154 86 86 154 ],[3.480000e-001 3.960000e-001 3.400000e-001 ]);
      | patch([211 211 215 215 ],[74 6 6 74 ],[2.240000e-001 2.480000e-001 2.200000e-001 ]);
      | patch([4 210 210 4 4 ],[0 0 240 240 0 ],[7.200000e-001 8.400000e-001 7.000000e-001 ]);
      | plot([4 210 210 4 4 ],[0 0 240 240 0 ]);
      |
      |
      | patch([40.25 83.6 113.6 143.6 173.6 113.6 70.25 40.25 ],[153.3 153.3 183.3 153.3 183.3 183.3 183.3 153.3 ],[1 1 1 ]);
      | patch([70.25 113.6 83.6 40.25 70.25 ],[123.3 123.3 153.3 153.3 123.3 ],[0.916 0.952 0.91 ]);
      | patch([40.25 83.6 113.6 70.25 40.25 ],[93.3 93.3 123.3 123.3 93.3 ],[1 1 1 ]);
      | patch([70.25 173.6 143.6 113.6 83.6 40.25 70.25 ],[63.3 63.3 93.3 63.3 93.3 93.3 63.3 ],[0.916 0.952 0.91 ]);
      | fprintf('','COMMENT: end icon graphics');
      | fprintf('','COMMENT: begin icon text');
      | color('black');port_label('input',1,'  data_tvalid  ');
      | color('black');port_label('input',2,'  data_tdata_data_in1  ');
      | color('black');port_label('input',3,'  data_tdata_data_in0  ');
      | color('black');port_label('input',4,'  dstat_tvalid  ');
      | color('black');port_label('input',5,'  dstat_tdata_ber_range  ');
      | color('black');port_label('input',6,'  data_tready  ');
      | color('black');port_label('input',7,'  dstat_tready  ');
      | color('black');port_label('output',1,'  data_tready  ');
      | color('black');port_label('output',2,'  dstat_tready  ');
      | color('black');port_label('output',3,'  data_tvalid  ');
      | color('black');port_label('output',4,'  data_tdata_data  ');
      | color('black');port_label('output',5,'  dstat_tvalid  ');
      | color('black');port_label('output',6,'  dstat_tdata_ber  ');
      | fprintf('','COMMENT: end icon text');
      mask prompts: channels "Number of Channels"; viterbi_type_sgadvanced ""; viterbi_type ""; reduced_latency_sgadvanced ""; reduced_latency "Use Reduced Latency"; constraint_length "Constraint Length"; traceback_length "Traceback Length"; architecture_sgadvanced ""; architecture ""; best_state_sgadvanced ""; best_state "Use Best State"; best_state_width "Best State Width"; puncturing_sgadvanced ""; puncturing ""; soft_width "Soft Width"; coding_sgadvanced ""; coding ""; data_format_sgadvanced ""; data_format ""; output_rate0 "Output Rate 0"; convolution_code_0_radix "Convolution Code 0 Radix"; convolution0_code0 "Convolution 0 Code 0"; convolution0_code1 "Convolution 0 Code 1"; convolution0_code2 "Convolution 0 Code 2"; convolution0_code3 "Convolution 0 Code 3"; convolution0_code4 "Convolution 0 Code 4"; convolution0_code5 "Convolution 0 Code 5"; convolution0_code6 "Convolution 0 Code 6"; output_rate1 "Output Rate 1"; convolution_code_1_radix "Convolution Code 1 Radix"; convolution1_code0 "Convolution 1 Code 0"; convolution1_code1 "Convolution 1 Code 1"; convolution1_code2 "Convolution 1 Code 2"; convolution1_code3 "Convolution 1 Code 3"; convolution1_code4 "Convolution 1 Code 4"; convolution1_code5 "Convolution 1 Code 5"; convolution1_code6 "Convolution 1 Code 6"; ber_symbol_count_sgadvanced ""; ber_symbol_count "Use BER Symbol Count"; norm_sgadvanced ""; block_valid_sgadvanced ""; block_valid "Block Valid"; tready_sgadvanced ""; aclken_sgadvanced ""; aresetn_sgadvanced ""; trim_axipin_name "Display shortened port names"; ip_name ""; ip_version ""; dsptool_ready ""; ipcore_usecache ""; ipcore_useipmodelcache ""; wrapper_available ""; port_translation_map ""; structural_sim ""; has_advanced_control ""; sggui_pos ""; block_type ""; block_version ""; sg_icon_stat ""; sg_mask_display ""; sg_list_contents ""; sg_blockgui_xml ""
      mask help: Xilinx Viterbi Decoder 8.0
      mask init:
      | try
      |   tmp_gcb = gcb;
      |   tmp_gcbh = gcbh;
      |   if (strcmp('SysGenIndex',get_param(bdroot(tmp_gcbh),'tag')) && ~isempty(regexp(bdroot(tmp_gcb), '^xbs', 'once')))
      |     return;
      |   end;
      |   xlMungeMaskParams;
      |   block_config = 'sysgen:coregenimport_config';
      | 
      |   block_type='viterbi_v8_0';
      | 
      |   serialized_declarations = '{''aclken''=>''Bool'',''architecture''=>''String'',''aresetn''=>''Bool'',''ber_symbol_count''=>''Bool'',''best_state''=>''Bool'',''best_state_width''=>''Int'',''block_valid''=>''Bool'',''channels''=>''Int'',''coding''=>''String'',''constraint_length''=>''Int'',''convolution0_code0''=>''String'',''convolution0_code1''=>''String'',''convolution0_code2''=>''String'',''convolution0_code3''=>''String'',''convolution0_code4''=>''String'',''convolution0_code5''=>''String'',''convolution0_code6''=>''String'',''convolution1_code0''=>''String'',''convolution1_code1''=>''String'',''convolution1_code2''=>''String'',''convolution1_code3''=>''String'',''convolution1_code4''=>''String'',''convolution1_code5''=>''String'',''convolution1_code6''=>''String'',''convolution_code_0_radix''=>''String'',''convolution_code_1_radix''=>''String'',''data_format''=>''String'',''dsptool_ready''=>''Bool'',''ip_name''=>''String'',''ip_version''=>''String'',''ipcore_usecache''=>''Bool'',''ipcore_useipmodelcache''=>''Bool'',''norm''=>''Bool'',''output_rate0''=>''String'',''output_rate1''=>''String'',''port_translation_map''=>''String'',''puncturing''=>''String'',''reduced_latency''=>''Bool'',''soft_width''=>''Int'',''structural_sim''=>''Bool'',''traceback_length''=>''Int'',''tready''=>''Bool'',''trim_axipin_name''=>''Int'',''viterbi_type''=>''String'',''wrapper_available''=>''Bool'',''block_type''=>''String''}';
      |   ptable_ = xlblockprep(get_param(tmp_gcb, 'MaskWSVariables'));
      |   try
      |     xlBlockMoveCallback(tmp_gcbh);
      |   catch 
      |      clear global xl_updateicon_recursion_guard;
      |   end;
      | catch
      |   global dbgsysgen;
      |   if(~isempty(dbgsysgen) && dbgsysgen)
      |     e = regexprep(lasterr, '\n', '\nError: ');
      |     disp(['Error: While running MaskInit code on block ' tmp_gcb ': ' e]);
      |     error(e);
      |   end
      | end
      settings: CopyFcn=xlBlockMoveCallback(gcbh);  DeleteFcn=xlDestroyGui(gcbh);  ModelCloseFcn=xlDestroyGui(gcbh);  PreSaveFcn=xlBlockPreSaveCallback(gcbh);  PostSaveFcn=xlBlockPostSaveCallback(gcbh);  DestroyFcn=xlDestroyGui(gcbh);  OpenFcn=xlOpenGui(gcbh, 'viterbi_v8_0_gui.xml', @viterbi_v8_0_enablement, @xlipmagicaction)  CloseFcn=xlDestroyGui(gcbh);  MoveFcn=xlBlockMoveCallback(gcbh);
      mask Help: eval('');xlDoc('-book','sysgen','-topic','Viterbi_Decoder_8_0');
      mask StyleString: edit,edit,popup(Standard|Multi_Channel|Trellis_Mode|Dual_Decoder),edit,checkbox,edit,edit,edit,popup(Parallel|Serial),edit,checkbox,edit,edit,popup(None|External),edit,edit,popup(Soft_Coding|Hard_Coding),edit,popup(Signed_Magnitude|Offset_Binary),popup(2|3|4|5|6|7),popup(Binary|Octal|Decimal),edit,edit,edit,edit,edit,edit,edit,popup(2|3|4|5|6|7),popup(Binary|Octal|Decimal),edit,edit,edit,edit,edit,edit,edit,edit,checkbox,edit,checkbox,edit,checkbox,edit,checkbox,edit,checkbox,edit,checkbox,checkbox,edit,edit,edit,edit,edit,edit,edit,edit,edit,edit,edit,edit,edit,edit,edit,edit
      mask Display:
      | fprintf('','COMMENT: begin icon graphics');
      | patch([0 0 4 4 ],[237 143 143 237 ],[5.960000e-001 6.920000e-001 5.800000e-001 ]);
      | patch([0 0 4 4 ],[132 73 73 132 ],[4.720000e-001 5.440000e-001 4.600000e-001 ]);
      | patch([0 0 4 4 ],[62 38 38 62 ],[3.480000e-001 3.960000e-001 3.400000e-001 ]);
      | patch([0 0 4 4 ],[27 3 3 27 ],[2.240000e-001 2.480000e-001 2.200000e-001 ]);
      | patch([211 211 215 215 ],[234 206 206 234 ],[5.960000e-001 6.920000e-001 5.800000e-001 ]);
      | patch([211 211 215 215 ],[194 166 166 194 ],[4.720000e-001 5.440000e-001 4.600000e-001 ]);
      | patch([211 211 215 215 ],[154 86 86 154 ],[3.480000e-001 3.960000e-001 3.400000e-001 ]);
      | patch([211 211 215 215 ],[74 6 6 74 ],[2.240000e-001 2.480000e-001 2.200000e-001 ]);
      | patch([4 210 210 4 4 ],[0 0 240 240 0 ],[7.200000e-001 8.400000e-001 7.000000e-001 ]);
      | plot([4 210 210 4 4 ],[0 0 240 240 0 ]);
      | 
      | 
      | patch([40.25 83.6 113.6 143.6 173.6 113.6 70.25 40.25 ],[153.3 153.3 183.3 153.3 183.3 183.3 183.3 153.3 ],[1 1 1 ]);
      | patch([70.25 113.6 83.6 40.25 70.25 ],[123.3 123.3 153.3 153.3 123.3 ],[0.916 0.952 0.91 ]);
      | patch([40.25 83.6 113.6 70.25 40.25 ],[93.3 93.3 123.3 123.3 93.3 ],[1 1 1 ]);
      | patch([70.25 173.6 143.6 113.6 83.6 40.25 70.25 ],[63.3 63.3 93.3 63.3 93.3 93.3 63.3 ],[0.916 0.952 0.91 ]);
      | fprintf('','COMMENT: end icon graphics');
      | fprintf('','COMMENT: begin icon text');
      | color('black');port_label('input',1,'  data_tvalid  ');
      | color('black');port_label('input',2,'  data_tdata_data_in1  ');
      | color('black');port_label('input',3,'  data_tdata_data_in0  ');
      | color('black');port_label('input',4,'  dstat_tvalid  ');
      | color('black');port_label('input',5,'  dstat_tdata_ber_range  ');
      | color('black');port_label('input',6,'  data_tready  ');
      | color('black');port_label('input',7,'  dstat_tready  ');
      | color('black');port_label('output',1,'  data_tready  ');
      | color('black');port_label('output',2,'  dstat_tready  ');
      | color('black');port_label('output',3,'  data_tvalid  ');
      | color('black');port_label('output',4,'  data_tdata_data  ');
      | color('black');port_label('output',5,'  dstat_tvalid  ');
      | color('black');port_label('output',6,'  dstat_tdata_ber  ');
      | fprintf('','COMMENT: end icon text');
  "Viterbi Decoder v5_0 " : S-Function  LoadFcn=xlBlockLoadCallback(gcbh);  FunctionName=sysgen  Parameters=ptable_  EnableBusSupport=off  mask(Xilinx Viterbi Decoder Block){infoedit=Decodes convolutionally encoded data. Number of input ports equals the length of the convolution code array., clength=7, dual_decoding_sgadvanced=, dual_decoding=off, conv_codes=[7 7], conv_codes2=[117 127], tb_length=36, coding_sgadvanced=, coding=Soft, data_format_sgadvanced=, data_format=Signed Magnitude, has_ber_sgadvanced=, has_ber=off, ber_rate=20, has_norm_sgadvanced=, has_norm=off, rst_sgadvanced=, rst=off, en_sgadvanced=, en=off, puncturing_sgadvanced=, puncturing=off, best_state_sgadvanced=, best_state=off, best_state_wr_sgadvanced=, best_state_wr=0, dbl_ovrd_sgadvanced=, dbl_ovrd=off, architecture_sgadvanced=, architecture=Parallel, optimization_sgadvanced=, optimization=Area, red_latency_sgadvanced=, red_latency=off, use_rpm_sgadvanced=, use_rpm=on, xl_use_area_sgadvanced=, xl_use_area=off, xl_area=[0,0,0,0,0,0,0], version=5, has_advanced_control=0, sggui_pos=-1,-1,-1,-1, block_type=viterbiv5, block_version=, sg_icon_stat=60,56,-1,-1,white,green,0,07734,right,,[ ],[ ], sg_mask_display=|, sg_list_contents=, sg_blockgui_xml=}
      mask sg_mask_display=|
      | fprintf('','COMMENT: begin icon graphics');
      | patch([0 60 60 0 0 ],[0 0 56 56 0 ],[0.72 0.84 0.7 ]);
      | plot([0 60 60 0 0 ],[0 0 56 56 0 ]);
      | patch([12.2 23.76 31.76 39.76 47.76 31.76 20.2 12.2 ],[36.88 36.88 44.88 36.88 44.88 44.88 44.88 36.88 ],[1 1 1 ]);
      | patch([20.2 31.76 23.76 12.2 20.2 ],[28.88 28.88 36.88 36.88 28.88 ],[0.916 0.952 0.91 ]);
      | patch([12.2 23.76 31.76 20.2 12.2 ],[20.88 20.88 28.88 28.88 20.88 ],[1 1 1 ]);
      | patch([20.2 47.76 39.76 31.76 23.76 12.2 20.2 ],[12.88 12.88 20.88 12.88 20.88 20.88 12.88 ],[0.916 0.952 0.91 ]);
      | fprintf('','COMMENT: end icon graphics');
      | fprintf('','COMMENT: begin icon text');
      | fprintf('','COMMENT: end icon text');
      mask prompts: infoedit ""; clength "Constraint length"; dual_decoding_sgadvanced ""; dual_decoding "Use dual decoder"; conv_codes "Convolution code array 1 (octal)"; conv_codes2 "Convolution code array 2 (octal)"; tb_length "Traceback length"; coding_sgadvanced ""; data_format_sgadvanced ""; data_format "Data format"; has_ber_sgadvanced ""; has_ber "Provide bit error rate port"; ber_rate "Number of input samples for error count"; has_norm_sgadvanced ""; has_norm "Provide normalization port"; rst_sgadvanced ""; rst "Provide synchronous reset port"; en_sgadvanced ""; en "Provide enable port"; puncturing_sgadvanced ""; puncturing "Use external puncturing"; best_state_sgadvanced ""; best_state "Use best state"; best_state_wr_sgadvanced ""; best_state_wr "Width reduction"; dbl_ovrd_sgadvanced ""; dbl_ovrd "Override with doubles"; architecture_sgadvanced ""; architecture "Architecture type"; optimization_sgadvanced ""; red_latency_sgadvanced ""; red_latency "Reduce latency"; use_rpm_sgadvanced ""; use_rpm "Use core placement information"; xl_use_area_sgadvanced ""; xl_use_area "Define FPGA area for resource estimation"; xl_area "FPGA area [slices, FFs, BRAMs, LUTs, IOBs, emb. mults, TBUFs]"; version ""; has_advanced_control ""; sggui_pos ""; block_type ""; block_version ""; sg_icon_stat ""; sg_mask_display ""; sg_list_contents ""; sg_blockgui_xml ""
      mask help: Decodes convolutionally encoded data. Number of input ports equals the length of the convolution code array.
      mask init:
      | try
      |   tmp_gcb = gcb;
      |   tmp_gcbh = gcbh;
      |   if (strcmp('SysGenIndex',get_param(bdroot(tmp_gcbh),'tag')) && ~isempty(regexp(bdroot(tmp_gcb), '^xbs', 'once')))
      |     return;
      |   end;
      |   xlMungeMaskParams;
      |   block_config = 'sysgen_blockset:Removed_config';
      | 
      |   block_type='viterbiv5';
      | nport = get_param(gcbh, 'ports');
      | nin = nport(1);
      | nout = nport(2);
      | 
      |   serialized_declarations = '{''architecture''=>''Int'',''ber_rate''=>''Int'',''best_state''=>''Int'',''best_state_wr''=>''Int'',''block_valid''=>''Int'',''clength''=>''Int'',''coding''=>''Int'',''conv_codes''=>''IntVector'',''conv_codes2''=>''IntVector'',''data_format''=>''Int'',''dual_decoding''=>''Int'',''en''=>''Int'',''has_ber''=>''Int'',''has_norm''=>''Int'',''optimization''=>''Int'',''puncturing''=>''Int'',''red_latency''=>''Int'',''rst''=>''Int'',''tb_length''=>''Int'',''version''=>''Int'',''block_type''=>''String'',''nin''=>''Double'',''nout''=>''Double''}';
      |   ptable_ = xlblockprep(get_param(tmp_gcb, 'MaskWSVariables'));
      |   try
      |     xlBlockMoveCallback(tmp_gcbh);
      |   catch 
      |      clear global xl_updateicon_recursion_guard;
      |   end;
      | catch
      |   global dbgsysgen;
      |   if(~isempty(dbgsysgen) && dbgsysgen)
      |     e = regexprep(lasterr, '\n', '\nError: ');
      |     disp(['Error: While running MaskInit code on block ' tmp_gcb ': ' e]);
      |     error(e);
      |   end
      | end
      settings: CopyFcn=xlBlockMoveCallback(gcbh);  DeleteFcn=xlDestroyGui(gcbh);  ModelCloseFcn=xlDestroyGui(gcbh);  PreSaveFcn=xlBlockPreSaveCallback(gcbh);  PostSaveFcn=xlBlockPostSaveCallback(gcbh);  DestroyFcn=xlDestroyGui(gcbh);  OpenFcn=xlOpenGui(gcbh, 'viterbi_gui.xml', @xlremovedenablement, -1)  CloseFcn=xlDestroyGui(gcbh);  MoveFcn=xlBlockMoveCallback(gcbh);
      mask Help: eval('');xlDoc('-book','sysgen','-topic','Viterbi_Decoder_v5_0');
      mask StyleString: edit,edit,edit,checkbox,edit,edit,edit,edit,popup(Soft|Hard),edit,popup(Signed Magnitude|Offset Binary),edit,checkbox,edit,edit,checkbox,edit,checkbox,edit,checkbox,edit,checkbox,edit,checkbox,edit,popup(0|1|2|3),edit,checkbox,edit,popup(Parallel|Serial),edit,popup(Area|Speed),edit,checkbox,edit,checkbox,edit,checkbox,edit,edit,edit,edit,edit,edit,edit,edit,edit,edit
      mask Display:
      | fprintf('','COMMENT: begin icon graphics');
      | patch([0 60 60 0 0 ],[0 0 56 56 0 ],[0.72 0.84 0.7 ]);
      | plot([0 60 60 0 0 ],[0 0 56 56 0 ]);
      | patch([12.2 23.76 31.76 39.76 47.76 31.76 20.2 12.2 ],[36.88 36.88 44.88 36.88 44.88 44.88 44.88 36.88 ],[1 1 1 ]);
      | patch([20.2 31.76 23.76 12.2 20.2 ],[28.88 28.88 36.88 36.88 28.88 ],[0.916 0.952 0.91 ]);
      | patch([12.2 23.76 31.76 20.2 12.2 ],[20.88 20.88 28.88 28.88 20.88 ],[1 1 1 ]);
      | patch([20.2 47.76 39.76 31.76 23.76 12.2 20.2 ],[12.88 12.88 20.88 12.88 20.88 20.88 12.88 ],[0.916 0.952 0.91 ]);
      | fprintf('','COMMENT: end icon graphics');
      | fprintf('','COMMENT: begin icon text');
      | fprintf('','COMMENT: end icon text');
  "Viterbi Decoder v6_0 " : S-Function  LoadFcn=xlBlockLoadCallback(gcbh);  FunctionName=sysgen  Parameters=ptable_  EnableBusSupport=off  mask(Xilinx Viterbi Decoder Block){infoedit=Decodes convolutionally encoded data. Number of input ports equals the length of the convolution code array., clength=7, dual_decoding_sgadvanced=, dual_decoding=off, conv_codes=[7 7], conv_codes2=[117 127], tb_length=36, coding_sgadvanced=, coding=Soft, data_format_sgadvanced=, data_format=Signed Magnitude, has_ber_sgadvanced=, has_ber=off, ber_rate=20, has_norm_sgadvanced=, has_norm=off, rst_sgadvanced=, rst=off, en_sgadvanced=, en=off, puncturing_sgadvanced=, puncturing=off, best_state_sgadvanced=, best_state=off, best_state_wr_sgadvanced=, best_state_wr=0, dbl_ovrd_sgadvanced=, dbl_ovrd=off, architecture_sgadvanced=, architecture=Parallel, optimization_sgadvanced=, optimization=Area, red_latency_sgadvanced=, red_latency=off, use_rpm_sgadvanced=, use_rpm=on, xl_use_area_sgadvanced=, xl_use_area=off, xl_area=[0,0,0,0,0,0,0], version=6, has_advanced_control=0, sggui_pos=-1,-1,-1,-1, block_type=viterbiv6, block_version=, sg_icon_stat=60,56,-1,-1,white,green,0,07734,right,,[ ],[ ], sg_mask_display=|, sg_list_contents=, sg_blockgui_xml=}
      mask sg_mask_display=|
      | fprintf('','COMMENT: begin icon graphics');
      | patch([0 60 60 0 0 ],[0 0 56 56 0 ],[0.72 0.84 0.7 ]);
      | plot([0 60 60 0 0 ],[0 0 56 56 0 ]);
      | patch([12.2 23.76 31.76 39.76 47.76 31.76 20.2 12.2 ],[36.88 36.88 44.88 36.88 44.88 44.88 44.88 36.88 ],[1 1 1 ]);
      | patch([20.2 31.76 23.76 12.2 20.2 ],[28.88 28.88 36.88 36.88 28.88 ],[0.916 0.952 0.91 ]);
      | patch([12.2 23.76 31.76 20.2 12.2 ],[20.88 20.88 28.88 28.88 20.88 ],[1 1 1 ]);
      | patch([20.2 47.76 39.76 31.76 23.76 12.2 20.2 ],[12.88 12.88 20.88 12.88 20.88 20.88 12.88 ],[0.916 0.952 0.91 ]);
      | fprintf('','COMMENT: end icon graphics');
      | fprintf('','COMMENT: begin icon text');
      | fprintf('','COMMENT: end icon text');
      mask prompts: infoedit ""; clength "Constraint length"; dual_decoding_sgadvanced ""; dual_decoding "Use dual decoder"; conv_codes "Convolution code array 1 (octal)"; conv_codes2 "Convolution code array 2 (octal)"; tb_length "Traceback length"; coding_sgadvanced ""; data_format_sgadvanced ""; data_format "Data format"; has_ber_sgadvanced ""; has_ber "Provide bit error rate port"; ber_rate "Number of input samples for error count"; has_norm_sgadvanced ""; has_norm "Provide normalization port"; rst_sgadvanced ""; rst "Provide synchronous reset port"; en_sgadvanced ""; en "Provide enable port"; puncturing_sgadvanced ""; puncturing "Use external puncturing"; best_state_sgadvanced ""; best_state "Use best state"; best_state_wr_sgadvanced ""; best_state_wr "Width reduction"; dbl_ovrd_sgadvanced ""; dbl_ovrd "Override with doubles"; architecture_sgadvanced ""; architecture "Architecture type"; optimization_sgadvanced ""; red_latency_sgadvanced ""; red_latency "Reduce latency"; use_rpm_sgadvanced ""; use_rpm "Use core placement information"; xl_use_area_sgadvanced ""; xl_use_area "Define FPGA area for resource estimation"; xl_area "FPGA area [slices, FFs, BRAMs, LUTs, IOBs, emb. mults, TBUFs]"; version ""; has_advanced_control ""; sggui_pos ""; block_type ""; block_version ""; sg_icon_stat ""; sg_mask_display ""; sg_list_contents ""; sg_blockgui_xml ""
      mask help: Decodes convolutionally encoded data. Number of input ports equals the length of the convolution code array.
      mask init:
      | try
      |   tmp_gcb = gcb;
      |   tmp_gcbh = gcbh;
      |   if (strcmp('SysGenIndex',get_param(bdroot(tmp_gcbh),'tag')) && ~isempty(regexp(bdroot(tmp_gcb), '^xbs', 'once')))
      |     return;
      |   end;
      |   xlMungeMaskParams;
      |   block_config = 'sysgen_blockset:Removed_config';
      | 
      |   block_type='viterbiv6';
      | nport = get_param(gcbh, 'ports');
      | nin = nport(1);
      | nout = nport(2);
      | 
      |   serialized_declarations = '{''architecture''=>''Int'',''ber_rate''=>''Int'',''best_state''=>''Int'',''best_state_wr''=>''Int'',''block_valid''=>''Int'',''clength''=>''Int'',''coding''=>''Int'',''conv_codes''=>''IntVector'',''conv_codes2''=>''IntVector'',''data_format''=>''Int'',''dual_decoding''=>''Int'',''en''=>''Int'',''has_ber''=>''Int'',''has_norm''=>''Int'',''optimization''=>''Int'',''puncturing''=>''Int'',''red_latency''=>''Int'',''rst''=>''Int'',''tb_length''=>''Int'',''version''=>''Int'',''block_type''=>''String'',''nin''=>''Double'',''nout''=>''Double''}';
      |   ptable_ = xlblockprep(get_param(tmp_gcb, 'MaskWSVariables'));
      |   try
      |     xlBlockMoveCallback(tmp_gcbh);
      |   catch 
      |      clear global xl_updateicon_recursion_guard;
      |   end;
      | catch
      |   global dbgsysgen;
      |   if(~isempty(dbgsysgen) && dbgsysgen)
      |     e = regexprep(lasterr, '\n', '\nError: ');
      |     disp(['Error: While running MaskInit code on block ' tmp_gcb ': ' e]);
      |     error(e);
      |   end
      | end
      settings: CopyFcn=xlBlockMoveCallback(gcbh);  DeleteFcn=xlDestroyGui(gcbh);  ModelCloseFcn=xlDestroyGui(gcbh);  PreSaveFcn=xlBlockPreSaveCallback(gcbh);  PostSaveFcn=xlBlockPostSaveCallback(gcbh);  DestroyFcn=xlDestroyGui(gcbh);  OpenFcn=xlOpenGui(gcbh, 'viterbiv6_gui.xml', @xlremovedenablement, -1)  CloseFcn=xlDestroyGui(gcbh);  MoveFcn=xlBlockMoveCallback(gcbh);
      mask Help: eval('');xlDoc('-book','sysgen','-topic','Viterbi_Decoder_v6_0');
      mask StyleString: edit,edit,edit,checkbox,edit,edit,edit,edit,popup(Soft|Hard),edit,popup(Signed Magnitude|Offset Binary),edit,checkbox,edit,edit,checkbox,edit,checkbox,edit,checkbox,edit,checkbox,edit,checkbox,edit,popup(0|1|2|3),edit,checkbox,edit,popup(Parallel|Serial),edit,popup(Area|Speed),edit,checkbox,edit,checkbox,edit,checkbox,edit,edit,edit,edit,edit,edit,edit,edit,edit,edit
      mask Display:
      | fprintf('','COMMENT: begin icon graphics');
      | patch([0 60 60 0 0 ],[0 0 56 56 0 ],[0.72 0.84 0.7 ]);
      | plot([0 60 60 0 0 ],[0 0 56 56 0 ]);
      | patch([12.2 23.76 31.76 39.76 47.76 31.76 20.2 12.2 ],[36.88 36.88 44.88 36.88 44.88 44.88 44.88 36.88 ],[1 1 1 ]);
      | patch([20.2 31.76 23.76 12.2 20.2 ],[28.88 28.88 36.88 36.88 28.88 ],[0.916 0.952 0.91 ]);
      | patch([12.2 23.76 31.76 20.2 12.2 ],[20.88 20.88 28.88 28.88 20.88 ],[1 1 1 ]);
      | patch([20.2 47.76 39.76 31.76 23.76 12.2 20.2 ],[12.88 12.88 20.88 12.88 20.88 20.88 12.88 ],[0.916 0.952 0.91 ]);
      | fprintf('','COMMENT: end icon graphics');
      | fprintf('','COMMENT: begin icon text');
      | fprintf('','COMMENT: end icon text');
  "Viterbi Decoder v6_1 " : S-Function  LoadFcn=xlBlockLoadCallback(gcbh);  FunctionName=sysgen  Parameters=ptable_  EnableBusSupport=off  mask(Xilinx Viterbi Decoder Block){infoedit=Decodes convolutionally encoded data. Number of input ports equals the length of the convolution code array., clength=7, dual_decoding_sgadvanced=, dual_decoding=off, conv_codes=[7 7], conv_codes2=[117 127], tb_length=36, coding_sgadvanced=, coding=Soft, data_format_sgadvanced=, data_format=Signed Magnitude, has_ber_sgadvanced=, has_ber=off, ber_rate=20, has_norm_sgadvanced=, has_norm=off, rst_sgadvanced=, rst=off, en_sgadvanced=, en=off, puncturing_sgadvanced=, puncturing=off, best_state_sgadvanced=, best_state=off, best_state_wr_sgadvanced=, best_state_wr=3, dbl_ovrd_sgadvanced=, dbl_ovrd=off, architecture_sgadvanced=, architecture=Parallel, optimization_sgadvanced=, optimization=Area, red_latency_sgadvanced=, red_latency=off, use_rpm_sgadvanced=, use_rpm=on, xl_use_area_sgadvanced=, xl_use_area=off, xl_area=[0,0,0,0,0,0,0], version=61, has_advanced_control=0, sggui_pos=-1,-1,-1,-1, block_type=viterbiv61, block_version=, sg_icon_stat=60,56,3,2,white,green,0,eb727c6b,right,,[ ],[ ], sg_mask_display=|, sg_list_contents=, sg_blockgui_xml=}
      mask sg_mask_display=|
      | fprintf('','COMMENT: begin icon graphics');
      | patch([0 60 60 0 0 ],[0 0 56 56 0 ],[0.72 0.84 0.7 ]);
      | plot([0 60 60 0 0 ],[0 0 56 56 0 ]);
      | patch([12.2 23.76 31.76 39.76 47.76 31.76 20.2 12.2 ],[36.88 36.88 44.88 36.88 44.88 44.88 44.88 36.88 ],[1 1 1 ]);
      | patch([20.2 31.76 23.76 12.2 20.2 ],[28.88 28.88 36.88 36.88 28.88 ],[0.916 0.952 0.91 ]);
      | patch([12.2 23.76 31.76 20.2 12.2 ],[20.88 20.88 28.88 28.88 20.88 ],[1 1 1 ]);
      | patch([20.2 47.76 39.76 31.76 23.76 12.2 20.2 ],[12.88 12.88 20.88 12.88 20.88 20.88 12.88 ],[0.916 0.952 0.91 ]);
      | fprintf('','COMMENT: end icon graphics');
      | fprintf('','COMMENT: begin icon text');
      | color('black');port_label('input',1,'din1');
      | color('black');port_label('input',2,'din2');
      | color('black');port_label('input',3,'vin');
      | color('black');port_label('output',1,'dout');
      | color('black');port_label('output',2,'vout');
      | fprintf('','COMMENT: end icon text');
      mask prompts: infoedit ""; clength "Constraint length"; dual_decoding_sgadvanced ""; dual_decoding "Use dual decoder"; conv_codes "Convolution code array 1 (octal)"; conv_codes2 "Convolution code array 2 (octal)"; tb_length "Traceback length"; coding_sgadvanced ""; data_format_sgadvanced ""; data_format "Data format"; has_ber_sgadvanced ""; has_ber "Provide bit error rate port"; ber_rate "Number of input samples for error count"; has_norm_sgadvanced ""; has_norm "Provide normalization port"; rst_sgadvanced ""; rst "Provide synchronous reset port"; en_sgadvanced ""; en "Provide enable port"; puncturing_sgadvanced ""; puncturing "Use external puncturing"; best_state_sgadvanced ""; best_state "Use best state"; best_state_wr_sgadvanced ""; best_state_wr "Width reduction"; dbl_ovrd_sgadvanced ""; dbl_ovrd "Override with doubles"; architecture_sgadvanced ""; architecture "Architecture type"; optimization_sgadvanced ""; red_latency_sgadvanced ""; red_latency "Reduce latency"; use_rpm_sgadvanced ""; use_rpm "Use core placement information"; xl_use_area_sgadvanced ""; xl_use_area "Define FPGA area for resource estimation"; xl_area "FPGA area [slices, FFs, BRAMs, LUTs, IOBs, emb. mults, TBUFs]"; version ""; has_advanced_control ""; sggui_pos ""; block_type ""; block_version ""; sg_icon_stat ""; sg_mask_display ""; sg_list_contents ""; sg_blockgui_xml ""
      mask help: Decodes convolutionally encoded data. Number of input ports equals the length of the convolution code array.
      mask init:
      | try
      |   tmp_gcb = gcb;
      |   tmp_gcbh = gcbh;
      |   if (strcmp('SysGenIndex',get_param(bdroot(tmp_gcbh),'tag')) && ~isempty(regexp(bdroot(tmp_gcb), '^xbs', 'once')))
      |     return;
      |   end;
      |   xlMungeMaskParams;
      |   block_config = 'sysgen_blockset:Viterbi_config';
      | 
      |   block_type='viterbiv61';
      | 
      |   serialized_declarations = '{''architecture''=>''Int'',''ber_rate''=>''Int'',''best_state''=>''Int'',''best_state_wr''=>''Int'',''block_valid''=>''Int'',''clength''=>''Int'',''coding''=>''Int'',''conv_codes''=>''IntVector'',''conv_codes2''=>''IntVector'',''data_format''=>''Int'',''dual_decoding''=>''Int'',''en''=>''Int'',''has_ber''=>''Int'',''has_norm''=>''Int'',''optimization''=>''Int'',''puncturing''=>''Int'',''red_latency''=>''Int'',''rst''=>''Int'',''tb_length''=>''Int'',''version''=>''Int'',''block_type''=>''String''}';
      |   ptable_ = xlblockprep(get_param(tmp_gcb, 'MaskWSVariables'));
      |   try
      |     xlBlockMoveCallback(tmp_gcbh);
      |   catch 
      |      clear global xl_updateicon_recursion_guard;
      |   end;
      | catch
      |   global dbgsysgen;
      |   if(~isempty(dbgsysgen) && dbgsysgen)
      |     e = regexprep(lasterr, '\n', '\nError: ');
      |     disp(['Error: While running MaskInit code on block ' tmp_gcb ': ' e]);
      |     error(e);
      |   end
      | end
      settings: CopyFcn=xlBlockMoveCallback(gcbh);  DeleteFcn=xlDestroyGui(gcbh);  ModelCloseFcn=xlDestroyGui(gcbh);  PreSaveFcn=xlBlockPreSaveCallback(gcbh);  PostSaveFcn=xlBlockPostSaveCallback(gcbh);  DestroyFcn=xlDestroyGui(gcbh);  OpenFcn=xlOpenGui(gcbh, 'viterbiv61_gui.xml', @viterbienablement, -1)  CloseFcn=xlDestroyGui(gcbh);  MoveFcn=xlBlockMoveCallback(gcbh);
      mask Help: eval('');xlDoc('-book','sysgen','-topic','Viterbi_Decoder_v6_1');
      mask StyleString: edit,edit,edit,checkbox,edit,edit,edit,edit,popup(Soft|Hard),edit,popup(Signed Magnitude|Offset Binary),edit,checkbox,edit,edit,checkbox,edit,checkbox,edit,checkbox,edit,checkbox,edit,checkbox,edit,popup(3|4|5|6|7|8),edit,checkbox,edit,popup(Parallel|Serial),edit,popup(Area|Speed),edit,checkbox,edit,checkbox,edit,checkbox,edit,edit,edit,edit,edit,edit,edit,edit,edit,edit
      mask Display:
      | fprintf('','COMMENT: begin icon graphics');
      | patch([0 60 60 0 0 ],[0 0 56 56 0 ],[0.72 0.84 0.7 ]);
      | plot([0 60 60 0 0 ],[0 0 56 56 0 ]);
      | patch([12.2 23.76 31.76 39.76 47.76 31.76 20.2 12.2 ],[36.88 36.88 44.88 36.88 44.88 44.88 44.88 36.88 ],[1 1 1 ]);
      | patch([20.2 31.76 23.76 12.2 20.2 ],[28.88 28.88 36.88 36.88 28.88 ],[0.916 0.952 0.91 ]);
      | patch([12.2 23.76 31.76 20.2 12.2 ],[20.88 20.88 28.88 28.88 20.88 ],[1 1 1 ]);
      | patch([20.2 47.76 39.76 31.76 23.76 12.2 20.2 ],[12.88 12.88 20.88 12.88 20.88 20.88 12.88 ],[0.916 0.952 0.91 ]);
      | fprintf('','COMMENT: end icon graphics');
      | fprintf('','COMMENT: begin icon text');
      | color('black');port_label('input',1,'din1');
      | color('black');port_label('input',2,'din2');
      | color('black');port_label('input',3,'vin');
      | color('black');port_label('output',1,'dout');
      | color('black');port_label('output',2,'vout');
      | fprintf('','COMMENT: end icon text');
  WaveScope : S-Function  InitFcn=xlRegisterHandles(gcbh);  StopFcn=|  FunctionName=xlpermissive  Parameters=''  EnableBusSupport=off  mask(Xilinx WaveScope Block){infoedit=WaveScope, ShowPortLabels=, has_advanced_control=0, sggui_pos=-1,-1,-1,-1, block_type=wavescope, block_version=, sg_icon_stat=71,62,-1,-1,blue,white,0,07734,right,,[ ],[ ], sg_mask_display=|, sg_list_contents=, sg_blockgui_xml=}
      | userdata=get_param(gcbh,'userdata');
      | if(isfield(userdata,'RunAtEndOfSim')&&strcmp(userdata.RunAtEndOfSim,'on'))
      |   xlWaveScope(gcbh);
      | end
      mask sg_mask_display=|
      | fprintf('','COMMENT: begin icon graphics');
      | patch([0 71 71 0 0 ],[0 0 62 62 0 ],[1 1 1 ]);
      | plot([0 71 71 0 0 ],[0 0 62 62 0 ]);
      | patch([17.2 28.76 36.76 44.76 52.76 36.76 25.2 17.2 ],[39.88 39.88 47.88 39.88 47.88 47.88 47.88 39.88 ],[0.839 0.874 0.937 ]);
      | patch([25.2 36.76 28.76 17.2 25.2 ],[31.88 31.88 39.88 39.88 31.88 ],[0.77 0.82 0.91 ]);
      | patch([17.2 28.76 36.76 25.2 17.2 ],[23.88 23.88 31.88 31.88 23.88 ],[0.839 0.874 0.937 ]);
      | patch([25.2 52.76 44.76 36.76 28.76 17.2 25.2 ],[15.88 15.88 23.88 15.88 23.88 23.88 15.88 ],[0.77 0.82 0.91 ]);
      | fprintf('','COMMENT: end icon graphics');
      | fprintf('','COMMENT: begin icon text');
      | fprintf('','COMMENT: end icon text');color('green');
      | plot([0,0.42,0.57,1]*w,[0.62, 0.62, 0.38,0.38]*h);
      | plot([0,0.42,0.57,1]*w,[0.38, 0.38, 0.62,0.62]*h);
      | color('red');
      | plot([0,0.3,0.3,0.47,0.47,1]*w,[0.15,0.15,0.3,0.3,0.15,0.15]*h);
      | color('black');
      | text(0.08*w,0.5*h,'Wave');
      | text(0.56*w,0.5*h,'Scope');
      mask prompts: infoedit ""; ShowPortLabels ""; has_advanced_control ""; sggui_pos ""; block_type ""; block_version ""; sg_icon_stat ""; sg_mask_display ""; sg_list_contents ""; sg_blockgui_xml ""
      mask help: WaveScope
      mask init:
      | try
      |   tmp_gcb = gcb;
      |   tmp_gcbh = gcbh;
      |   xlMungeMaskParams;
      | 
      |   block_type='wavescope';
      | 
      |   serialized_declarations = '{''block_type''=>''String''}';
      |   xlwavescope_init();
      |   ptable_ = xlblockprep(get_param(tmp_gcb, 'MaskWSVariables'));
      |   try
      |     xlBlockMoveCallback(tmp_gcbh);
      |   catch 
      |      clear global xl_updateicon_recursion_guard;
      |   end;
      | catch
      |   global dbgsysgen;
      |   if(~isempty(dbgsysgen) && dbgsysgen)
      |     e = regexprep(lasterr, '\n', '\nError: ');
      |     disp(['Error: While running MaskInit code on block ' tmp_gcb ': ' e]);
      |     error(e);
      |   end
      | end
      settings: CopyFcn=xlWaveScopeCopyFcn(gcbh);  PreSaveFcn=xlRegisterHandles(gcbh);  OpenFcn=xlWaveScope(gcbh);  MoveFcn=xlBlockMoveCallback(gcbh);
      settings: DeleteFcn=|
      | fig_name = [ get_param(gcbh,'Parent') , '/', get_param(gcbh,'Name') ];
      | scopehandle = findobj('Name',fig_name);
      | if scopehandle
      |   close(scopehandle);
      | end
      settings: ModelCloseFcn=|
      | fig_name = [ get_param(gcbh,'Parent') , '/', get_param(gcbh,'Name') ];
      | scopehandle = findobj('Name',fig_name);
      | if scopehandle
      |   close(scopehandle);
      | end
      settings: DestroyFcn=|
      | fig_name = [ get_param(gcbh,'Parent') , '/', get_param(gcbh,'Name') ];
      | scopehandle = findobj('Name',fig_name);
      | if scopehandle
      |   close(scopehandle);
      | end
      mask Help: eval('');xlDoc('-book','sysgen','-topic','WaveScope');
      mask Display:
      | fprintf('','COMMENT: begin icon graphics');
      | patch([0 71 71 0 0 ],[0 0 62 62 0 ],[1 1 1 ]);
      | plot([0 71 71 0 0 ],[0 0 62 62 0 ]);
      | patch([17.2 28.76 36.76 44.76 52.76 36.76 25.2 17.2 ],[39.88 39.88 47.88 39.88 47.88 47.88 47.88 39.88 ],[0.839 0.874 0.937 ]);
      | patch([25.2 36.76 28.76 17.2 25.2 ],[31.88 31.88 39.88 39.88 31.88 ],[0.77 0.82 0.91 ]);
      | patch([17.2 28.76 36.76 25.2 17.2 ],[23.88 23.88 31.88 31.88 23.88 ],[0.839 0.874 0.937 ]);
      | patch([25.2 52.76 44.76 36.76 28.76 17.2 25.2 ],[15.88 15.88 23.88 15.88 23.88 23.88 15.88 ],[0.77 0.82 0.91 ]);
      | fprintf('','COMMENT: end icon graphics');
      | fprintf('','COMMENT: begin icon text');
      | fprintf('','COMMENT: end icon text');color('green');
      | plot([0,0.42,0.57,1]*w,[0.62, 0.62, 0.38,0.38]*h);
      | plot([0,0.42,0.57,1]*w,[0.38, 0.38, 0.62,0.62]*h);
      | color('red');
      | plot([0,0.3,0.3,0.47,0.47,1]*w,[0.15,0.15,0.3,0.3,0.15,0.15]*h);
      | color('black');
      | text(0.08*w,0.5*h,'Wave');
      | text(0.56*w,0.5*h,'Scope');
